simulink model "ami_fx_sbl_wide"  (R2012b)
(part 2 of 43)

      mask init:
      | gw_name = clear_name(gcb);
      | config.source = str2func('software_register_init');
      | config.toplevel = gcb;
      | xBlock( config, {io_dir, arith_type, bitwidth, bin_pt, ... 
      |     sample_period, gw_name, latency});
      mask TypeOptions io_dir: From Processor | To Processor
      mask TypeOptions arith_type: Unsigned | Signed  (2's comp)
  notused : xbsIndex_r4/Constant  const=0  gui_display_data_type=Fixed-point  arith_type=Boolean  n_bits=28  bin_pt=0  preci_type=Single  exp_width=8  frac_width=24  explicit_period=on  period=1  equ=P=C  opselect=C  inp2=PCIN>>17  opr=+  inp1=P  carry=CIN  dbl_ovrd=off  block_type=constant
  packetiser : Subsystem  mask{fft_bits=11}
      mask prompts: fft_bits "Number of frequencies (2^?)"
      mask help: Package 32 bit data into 64 bits and identify data as coming from antenna 0 or 1
  phase_invert1 : Subsystem
  phase_invert2 : Subsystem
  pipeline : Subsystem  AncestorBlock=casper_library_delays/pipeline  mask(pipeline){latency=1}
      mask help:
      | An explicitly laid-out delay line to avoid mapping to SRL16s
      | for use in pipelining to help achieve timing closure.
      mask init:
      | pipeline_init(gcb,'latency',latency);
      settings: AttributesFormatString=Latency = %<latency>
      mask Display:
      | port_label('input', 1, 'd');
      | port_label('output', 1, 'q');
      | disp(['Z^-', num2str(latency)]);
  pipeline1 : Subsystem  AncestorBlock=casper_library_delays/pipeline  mask(pipeline){latency=1}
      mask help:
      | An explicitly laid-out delay line to avoid mapping to SRL16s
      | for use in pipelining to help achieve timing closure.
      mask init:
      | pipeline_init(gcb,'latency',latency);
      settings: AttributesFormatString=Latency = %<latency>
      mask Display:
      | port_label('input', 1, 'd');
      | port_label('output', 1, 'q');
      | disp(['Z^-', num2str(latency)]);
  pipeline10 : Subsystem  AncestorBlock=casper_library_delays/pipeline  mask(pipeline){latency=3}
      mask help:
      | An explicitly laid-out delay line to avoid mapping to SRL16s
      | for use in pipelining to help achieve timing closure.
      mask init:
      | pipeline_init(gcb,'latency',latency);
      settings: AttributesFormatString=Latency = %<latency>
      mask Display:
      | port_label('input', 1, 'd');
      | port_label('output', 1, 'q');
      | disp(['Z^-', num2str(latency)]);
  pipeline100 : Subsystem  AncestorBlock=casper_library_delays/pipeline  mask(pipeline){latency=2}
      mask help:
      | An explicitly laid-out delay line to avoid mapping to SRL16s
      | for use in pipelining to help achieve timing closure.
      mask init:
      | pipeline_init(gcb,'latency',latency);
      settings: AttributesFormatString=Latency = %<latency>
      mask Display:
      | port_label('input', 1, 'd');
      | port_label('output', 1, 'q');
      | disp(['Z^-', num2str(latency)]);
  pipeline101 : Subsystem  AncestorBlock=casper_library_delays/pipeline  mask(pipeline){latency=2}
      mask help:
      | An explicitly laid-out delay line to avoid mapping to SRL16s
      | for use in pipelining to help achieve timing closure.
      mask init:
      | pipeline_init(gcb,'latency',latency);
      settings: AttributesFormatString=Latency = %<latency>
      mask Display:
      | port_label('input', 1, 'd');
      | port_label('output', 1, 'q');
      | disp(['Z^-', num2str(latency)]);
  pipeline102 : Subsystem  AncestorBlock=casper_library_delays/pipeline  mask(pipeline){latency=2}
      mask help:
      | An explicitly laid-out delay line to avoid mapping to SRL16s
      | for use in pipelining to help achieve timing closure.
      mask init:
      | pipeline_init(gcb,'latency',latency);
      settings: AttributesFormatString=Latency = %<latency>
      mask Display:
      | port_label('input', 1, 'd');
      | port_label('output', 1, 'q');
      | disp(['Z^-', num2str(latency)]);
  pipeline103 : Subsystem  AncestorBlock=casper_library_delays/pipeline  mask(pipeline){latency=2}
      mask help:
      | An explicitly laid-out delay line to avoid mapping to SRL16s
      | for use in pipelining to help achieve timing closure.
      mask init:
      | pipeline_init(gcb,'latency',latency);
      settings: AttributesFormatString=Latency = %<latency>
      mask Display:
      | port_label('input', 1, 'd');
      | port_label('output', 1, 'q');
      | disp(['Z^-', num2str(latency)]);
  pipeline104 : Subsystem  AncestorBlock=casper_library_delays/pipeline  mask(pipeline){latency=2}
      mask help:
      | An explicitly laid-out delay line to avoid mapping to SRL16s
      | for use in pipelining to help achieve timing closure.
      mask init:
      | pipeline_init(gcb,'latency',latency);
      settings: AttributesFormatString=Latency = %<latency>
      mask Display:
      | port_label('input', 1, 'd');
      | port_label('output', 1, 'q');
      | disp(['Z^-', num2str(latency)]);
  pipeline105 : Subsystem  AncestorBlock=casper_library_delays/pipeline  mask(pipeline){latency=2}
      mask help:
      | An explicitly laid-out delay line to avoid mapping to SRL16s
      | for use in pipelining to help achieve timing closure.
      mask init:
      | pipeline_init(gcb,'latency',latency);
      settings: AttributesFormatString=Latency = %<latency>
      mask Display:
      | port_label('input', 1, 'd');
      | port_label('output', 1, 'q');
      | disp(['Z^-', num2str(latency)]);
  pipeline106 : Subsystem  AncestorBlock=casper_library_delays/pipeline  mask(pipeline){latency=2}
      mask help:
      | An explicitly laid-out delay line to avoid mapping to SRL16s
      | for use in pipelining to help achieve timing closure.
      mask init:
      | pipeline_init(gcb,'latency',latency);
      settings: AttributesFormatString=Latency = %<latency>
      mask Display:
      | port_label('input', 1, 'd');
      | port_label('output', 1, 'q');
      | disp(['Z^-', num2str(latency)]);
  pipeline107 : Subsystem  AncestorBlock=casper_library_delays/pipeline  mask(pipeline){latency=2}
      mask help:
      | An explicitly laid-out delay line to avoid mapping to SRL16s
      | for use in pipelining to help achieve timing closure.
      mask init:
      | pipeline_init(gcb,'latency',latency);
      settings: AttributesFormatString=Latency = %<latency>
      mask Display:
      | port_label('input', 1, 'd');
      | port_label('output', 1, 'q');
      | disp(['Z^-', num2str(latency)]);
  pipeline108 : Subsystem  AncestorBlock=casper_library_delays/pipeline  mask(pipeline){latency=2}
      mask help:
      | An explicitly laid-out delay line to avoid mapping to SRL16s
      | for use in pipelining to help achieve timing closure.
      mask init:
      | pipeline_init(gcb,'latency',latency);
      settings: AttributesFormatString=Latency = %<latency>
      mask Display:
      | port_label('input', 1, 'd');
      | port_label('output', 1, 'q');
      | disp(['Z^-', num2str(latency)]);
  pipeline109 : Subsystem  AncestorBlock=casper_library_delays/pipeline  mask(pipeline){latency=2}
      mask help:
      | An explicitly laid-out delay line to avoid mapping to SRL16s
      | for use in pipelining to help achieve timing closure.
      mask init:
      | pipeline_init(gcb,'latency',latency);
      settings: AttributesFormatString=Latency = %<latency>
      mask Display:
      | port_label('input', 1, 'd');
      | port_label('output', 1, 'q');
      | disp(['Z^-', num2str(latency)]);
  pipeline11 : Subsystem  AncestorBlock=casper_library_delays/pipeline  mask(pipeline){latency=1}
      mask help:
      | An explicitly laid-out delay line to avoid mapping to SRL16s
      | for use in pipelining to help achieve timing closure.
      mask init:
      | pipeline_init(gcb,'latency',latency);
      settings: AttributesFormatString=Latency = %<latency>
      mask Display:
      | port_label('input', 1, 'd');
      | port_label('output', 1, 'q');
      | disp(['Z^-', num2str(latency)]);
  pipeline110 : Subsystem  AncestorBlock=casper_library_delays/pipeline  mask(pipeline){latency=2}
      mask help:
      | An explicitly laid-out delay line to avoid mapping to SRL16s
      | for use in pipelining to help achieve timing closure.
      mask init:
      | pipeline_init(gcb,'latency',latency);
      settings: AttributesFormatString=Latency = %<latency>
      mask Display:
      | port_label('input', 1, 'd');
      | port_label('output', 1, 'q');
      | disp(['Z^-', num2str(latency)]);
  pipeline12 : Subsystem  AncestorBlock=casper_library_delays/pipeline  mask(pipeline){latency=3}
      mask help:
      | An explicitly laid-out delay line to avoid mapping to SRL16s
      | for use in pipelining to help achieve timing closure.
      mask init:
      | pipeline_init(gcb,'latency',latency);
      settings: AttributesFormatString=Latency = %<latency>
      mask Display:
      | port_label('input', 1, 'd');
      | port_label('output', 1, 'q');
      | disp(['Z^-', num2str(latency)]);
  pipeline13 : Subsystem  AncestorBlock=casper_library_delays/pipeline  mask(pipeline){latency=1}
      mask help:
      | An explicitly laid-out delay line to avoid mapping to SRL16s
      | for use in pipelining to help achieve timing closure.
      mask init:
      | pipeline_init(gcb,'latency',latency);
      settings: AttributesFormatString=Latency = %<latency>
      mask Display:
      | port_label('input', 1, 'd');
      | port_label('output', 1, 'q');
      | disp(['Z^-', num2str(latency)]);
  pipeline14 : Subsystem  AncestorBlock=casper_library_delays/pipeline  mask(pipeline){latency=2}
      mask help:
      | An explicitly laid-out delay line to avoid mapping to SRL16s
      | for use in pipelining to help achieve timing closure.
      mask init:
      | pipeline_init(gcb,'latency',latency);
      settings: AttributesFormatString=Latency = %<latency>
      mask Display:
      | port_label('input', 1, 'd');
      | port_label('output', 1, 'q');
      | disp(['Z^-', num2str(latency)]);
  pipeline15 : Subsystem  AncestorBlock=casper_library_delays/pipeline  mask(pipeline){latency=2}
      mask help:
      | An explicitly laid-out delay line to avoid mapping to SRL16s
      | for use in pipelining to help achieve timing closure.
      mask init:
      | pipeline_init(gcb,'latency',latency);
      settings: AttributesFormatString=Latency = %<latency>
      mask Display:
      | port_label('input', 1, 'd');
      | port_label('output', 1, 'q');
      | disp(['Z^-', num2str(latency)]);
  pipeline16 : Subsystem  AncestorBlock=casper_library_delays/pipeline  mask(pipeline){latency=2}
      mask help:
      | An explicitly laid-out delay line to avoid mapping to SRL16s
      | for use in pipelining to help achieve timing closure.
      mask init:
      | pipeline_init(gcb,'latency',latency);
      settings: AttributesFormatString=Latency = %<latency>
      mask Display:
      | port_label('input', 1, 'd');
      | port_label('output', 1, 'q');
      | disp(['Z^-', num2str(latency)]);
  pipeline17 : Subsystem  AncestorBlock=casper_library_delays/pipeline  mask(pipeline){latency=2}
      mask help:
      | An explicitly laid-out delay line to avoid mapping to SRL16s
      | for use in pipelining to help achieve timing closure.
      mask init:
      | pipeline_init(gcb,'latency',latency);
      settings: AttributesFormatString=Latency = %<latency>
      mask Display:
      | port_label('input', 1, 'd');
      | port_label('output', 1, 'q');
      | disp(['Z^-', num2str(latency)]);
  pipeline18 : Subsystem  AncestorBlock=casper_library_delays/pipeline  mask(pipeline){latency=2}
      mask help:
      | An explicitly laid-out delay line to avoid mapping to SRL16s
      | for use in pipelining to help achieve timing closure.
      mask init:
      | pipeline_init(gcb,'latency',latency);
      settings: AttributesFormatString=Latency = %<latency>
      mask Display:
      | port_label('input', 1, 'd');
      | port_label('output', 1, 'q');
      | disp(['Z^-', num2str(latency)]);
  pipeline19 : Subsystem  AncestorBlock=casper_library_delays/pipeline  mask(pipeline){latency=1}
      mask help:
      | An explicitly laid-out delay line to avoid mapping to SRL16s
      | for use in pipelining to help achieve timing closure.
      mask init:
      | pipeline_init(gcb,'latency',latency);
      settings: AttributesFormatString=Latency = %<latency>
      mask Display:
      | port_label('input', 1, 'd');
      | port_label('output', 1, 'q');
      | disp(['Z^-', num2str(latency)]);
  pipeline2 : Subsystem  AncestorBlock=casper_library_delays/pipeline  mask(pipeline){latency=1}
      mask help:
      | An explicitly laid-out delay line to avoid mapping to SRL16s
      | for use in pipelining to help achieve timing closure.
      mask init:
      | pipeline_init(gcb,'latency',latency);
      settings: AttributesFormatString=Latency = %<latency>
      mask Display:
      | port_label('input', 1, 'd');
      | port_label('output', 1, 'q');
      | disp(['Z^-', num2str(latency)]);
  pipeline20 : Subsystem  AncestorBlock=casper_library_delays/pipeline  mask(pipeline){latency=1}
      mask help:
      | An explicitly laid-out delay line to avoid mapping to SRL16s
      | for use in pipelining to help achieve timing closure.
      mask init:
      | pipeline_init(gcb,'latency',latency);
      settings: AttributesFormatString=Latency = %<latency>
      mask Display:
      | port_label('input', 1, 'd');
      | port_label('output', 1, 'q');
      | disp(['Z^-', num2str(latency)]);
  pipeline21 : Subsystem  AncestorBlock=casper_library_delays/pipeline  mask(pipeline){latency=1}
      mask help:
      | An explicitly laid-out delay line to avoid mapping to SRL16s
      | for use in pipelining to help achieve timing closure.
      mask init:
      | pipeline_init(gcb,'latency',latency);
      settings: AttributesFormatString=Latency = %<latency>
      mask Display:
      | port_label('input', 1, 'd');
      | port_label('output', 1, 'q');
      | disp(['Z^-', num2str(latency)]);
  pipeline22 : Subsystem  AncestorBlock=casper_library_delays/pipeline  mask(pipeline){latency=1}
      mask help:
      | An explicitly laid-out delay line to avoid mapping to SRL16s
      | for use in pipelining to help achieve timing closure.
      mask init:
      | pipeline_init(gcb,'latency',latency);
      settings: AttributesFormatString=Latency = %<latency>
      mask Display:
      | port_label('input', 1, 'd');
      | port_label('output', 1, 'q');
      | disp(['Z^-', num2str(latency)]);
  pipeline23 : Subsystem  AncestorBlock=casper_library_delays/pipeline  mask(pipeline){latency=1}
      mask help:
      | An explicitly laid-out delay line to avoid mapping to SRL16s
      | for use in pipelining to help achieve timing closure.
      mask init:
      | pipeline_init(gcb,'latency',latency);
      settings: AttributesFormatString=Latency = %<latency>
      mask Display:
      | port_label('input', 1, 'd');
      | port_label('output', 1, 'q');
      | disp(['Z^-', num2str(latency)]);
  pipeline24 : Subsystem  AncestorBlock=casper_library_delays/pipeline  mask(pipeline){latency=1}
      mask help:
      | An explicitly laid-out delay line to avoid mapping to SRL16s
      | for use in pipelining to help achieve timing closure.
      mask init:
      | pipeline_init(gcb,'latency',latency);
      settings: AttributesFormatString=Latency = %<latency>
      mask Display:
      | port_label('input', 1, 'd');
      | port_label('output', 1, 'q');
      | disp(['Z^-', num2str(latency)]);
  pipeline25 : Subsystem  AncestorBlock=casper_library_delays/pipeline  mask(pipeline){latency=1}
      mask help:
      | An explicitly laid-out delay line to avoid mapping to SRL16s
      | for use in pipelining to help achieve timing closure.
      mask init:
      | pipeline_init(gcb,'latency',latency);
      settings: AttributesFormatString=Latency = %<latency>
      mask Display:
      | port_label('input', 1, 'd');
      | port_label('output', 1, 'q');
      | disp(['Z^-', num2str(latency)]);
  pipeline26 : Subsystem  AncestorBlock=casper_library_delays/pipeline  mask(pipeline){latency=1}
      mask help:
      | An explicitly laid-out delay line to avoid mapping to SRL16s
      | for use in pipelining to help achieve timing closure.
      mask init:
      | pipeline_init(gcb,'latency',latency);
      settings: AttributesFormatString=Latency = %<latency>
      mask Display:
      | port_label('input', 1, 'd');
      | port_label('output', 1, 'q');
      | disp(['Z^-', num2str(latency)]);
  pipeline27 : Subsystem  AncestorBlock=casper_library_delays/pipeline  mask(pipeline){latency=1}
      mask help:
      | An explicitly laid-out delay line to avoid mapping to SRL16s
      | for use in pipelining to help achieve timing closure.
      mask init:
      | pipeline_init(gcb,'latency',latency);
      settings: AttributesFormatString=Latency = %<latency>
      mask Display:
      | port_label('input', 1, 'd');
      | port_label('output', 1, 'q');
      | disp(['Z^-', num2str(latency)]);
  pipeline28 : Subsystem  AncestorBlock=casper_library_delays/pipeline  mask(pipeline){latency=1}
      mask help:
      | An explicitly laid-out delay line to avoid mapping to SRL16s
      | for use in pipelining to help achieve timing closure.
      mask init:
      | pipeline_init(gcb,'latency',latency);
      settings: AttributesFormatString=Latency = %<latency>
      mask Display:
      | port_label('input', 1, 'd');
      | port_label('output', 1, 'q');
      | disp(['Z^-', num2str(latency)]);
  pipeline29 : Subsystem  AncestorBlock=casper_library_delays/pipeline  mask(pipeline){latency=1}
      mask help:
      | An explicitly laid-out delay line to avoid mapping to SRL16s
      | for use in pipelining to help achieve timing closure.
      mask init:
      | pipeline_init(gcb,'latency',latency);
      settings: AttributesFormatString=Latency = %<latency>
      mask Display:
      | port_label('input', 1, 'd');
      | port_label('output', 1, 'q');
      | disp(['Z^-', num2str(latency)]);
  pipeline3 : Subsystem  AncestorBlock=casper_library_delays/pipeline  mask(pipeline){latency=1}
      mask help:
      | An explicitly laid-out delay line to avoid mapping to SRL16s
      | for use in pipelining to help achieve timing closure.
      mask init:
      | pipeline_init(gcb,'latency',latency);
      settings: AttributesFormatString=Latency = %<latency>
      mask Display:
      | port_label('input', 1, 'd');
      | port_label('output', 1, 'q');
      | disp(['Z^-', num2str(latency)]);
  pipeline30 : Subsystem  AncestorBlock=casper_library_delays/pipeline  mask(pipeline){latency=1}
      mask help:
      | An explicitly laid-out delay line to avoid mapping to SRL16s
      | for use in pipelining to help achieve timing closure.
      mask init:
      | pipeline_init(gcb,'latency',latency);
      settings: AttributesFormatString=Latency = %<latency>
      mask Display:
      | port_label('input', 1, 'd');
      | port_label('output', 1, 'q');
      | disp(['Z^-', num2str(latency)]);
  pipeline31 : Subsystem  AncestorBlock=casper_library_delays/pipeline  mask(pipeline){latency=1}
      mask help:
      | An explicitly laid-out delay line to avoid mapping to SRL16s
      | for use in pipelining to help achieve timing closure.
      mask init:
      | pipeline_init(gcb,'latency',latency);
      settings: AttributesFormatString=Latency = %<latency>
      mask Display:
      | port_label('input', 1, 'd');
      | port_label('output', 1, 'q');
      | disp(['Z^-', num2str(latency)]);
  pipeline32 : Subsystem  AncestorBlock=casper_library_delays/pipeline  mask(pipeline){latency=1}
      mask help:
      | An explicitly laid-out delay line to avoid mapping to SRL16s
      | for use in pipelining to help achieve timing closure.
      mask init:
      | pipeline_init(gcb,'latency',latency);
      settings: AttributesFormatString=Latency = %<latency>
      mask Display:
      | port_label('input', 1, 'd');
      | port_label('output', 1, 'q');
      | disp(['Z^-', num2str(latency)]);
  pipeline33 : Subsystem  AncestorBlock=casper_library_delays/pipeline  mask(pipeline){latency=1}
      mask help:
      | An explicitly laid-out delay line to avoid mapping to SRL16s
      | for use in pipelining to help achieve timing closure.
      mask init:
      | pipeline_init(gcb,'latency',latency);
      settings: AttributesFormatString=Latency = %<latency>
      mask Display:
      | port_label('input', 1, 'd');
      | port_label('output', 1, 'q');
      | disp(['Z^-', num2str(latency)]);
  pipeline34 : Subsystem  AncestorBlock=casper_library_delays/pipeline  mask(pipeline){latency=1}
      mask help:
      | An explicitly laid-out delay line to avoid mapping to SRL16s
      | for use in pipelining to help achieve timing closure.
      mask init:
      | pipeline_init(gcb,'latency',latency);
      settings: AttributesFormatString=Latency = %<latency>
      mask Display:
      | port_label('input', 1, 'd');
      | port_label('output', 1, 'q');
      | disp(['Z^-', num2str(latency)]);
  pipeline35 : Subsystem  AncestorBlock=casper_library_delays/pipeline  mask(pipeline){latency=1}
      mask help:
      | An explicitly laid-out delay line to avoid mapping to SRL16s
      | for use in pipelining to help achieve timing closure.
      mask init:
      | pipeline_init(gcb,'latency',latency);
      settings: AttributesFormatString=Latency = %<latency>
      mask Display:
      | port_label('input', 1, 'd');
      | port_label('output', 1, 'q');
      | disp(['Z^-', num2str(latency)]);
  pipeline36 : Subsystem  AncestorBlock=casper_library_delays/pipeline  mask(pipeline){latency=1}
      mask help:
      | An explicitly laid-out delay line to avoid mapping to SRL16s
      | for use in pipelining to help achieve timing closure.
      mask init:
      | pipeline_init(gcb,'latency',latency);
      settings: AttributesFormatString=Latency = %<latency>
      mask Display:
      | port_label('input', 1, 'd');
      | port_label('output', 1, 'q');
      | disp(['Z^-', num2str(latency)]);
  pipeline37 : Subsystem  AncestorBlock=casper_library_delays/pipeline  mask(pipeline){latency=1}
      mask help:
      | An explicitly laid-out delay line to avoid mapping to SRL16s
      | for use in pipelining to help achieve timing closure.
      mask init:
      | pipeline_init(gcb,'latency',latency);
      settings: AttributesFormatString=Latency = %<latency>
      mask Display:
      | port_label('input', 1, 'd');
      | port_label('output', 1, 'q');
      | disp(['Z^-', num2str(latency)]);
  pipeline38 : Subsystem  AncestorBlock=casper_library_delays/pipeline  mask(pipeline){latency=3}
      mask help:
      | An explicitly laid-out delay line to avoid mapping to SRL16s
      | for use in pipelining to help achieve timing closure.
      mask init:
      | pipeline_init(gcb,'latency',latency);
      settings: AttributesFormatString=Latency = %<latency>
      mask Display:
      | port_label('input', 1, 'd');
      | port_label('output', 1, 'q');
      | disp(['Z^-', num2str(latency)]);
  pipeline39 : Subsystem  AncestorBlock=casper_library_delays/pipeline  mask(pipeline){latency=1}
      mask help:
      | An explicitly laid-out delay line to avoid mapping to SRL16s
      | for use in pipelining to help achieve timing closure.
      mask init:
      | pipeline_init(gcb,'latency',latency);
      settings: AttributesFormatString=Latency = %<latency>
      mask Display:
      | port_label('input', 1, 'd');
      | port_label('output', 1, 'q');
      | disp(['Z^-', num2str(latency)]);
  pipeline4 : Subsystem  AncestorBlock=casper_library_delays/pipeline  mask(pipeline){latency=1}
      mask help:
      | An explicitly laid-out delay line to avoid mapping to SRL16s
      | for use in pipelining to help achieve timing closure.
      mask init:
      | pipeline_init(gcb,'latency',latency);
      settings: AttributesFormatString=Latency = %<latency>
      mask Display:
      | port_label('input', 1, 'd');
      | port_label('output', 1, 'q');
      | disp(['Z^-', num2str(latency)]);
  pipeline40 : Subsystem  AncestorBlock=casper_library_delays/pipeline  mask(pipeline){latency=1}
      mask help:
      | An explicitly laid-out delay line to avoid mapping to SRL16s
      | for use in pipelining to help achieve timing closure.
      mask init:
      | pipeline_init(gcb,'latency',latency);
      settings: AttributesFormatString=Latency = %<latency>
      mask Display:
      | port_label('input', 1, 'd');
      | port_label('output', 1, 'q');
      | disp(['Z^-', num2str(latency)]);
  pipeline41 : Subsystem  AncestorBlock=casper_library_delays/pipeline  mask(pipeline){latency=1}
      mask help:
      | An explicitly laid-out delay line to avoid mapping to SRL16s
      | for use in pipelining to help achieve timing closure.
      mask init:
      | pipeline_init(gcb,'latency',latency);
      settings: AttributesFormatString=Latency = %<latency>
      mask Display:
      | port_label('input', 1, 'd');
      | port_label('output', 1, 'q');
      | disp(['Z^-', num2str(latency)]);
  pipeline42 : Subsystem  AncestorBlock=casper_library_delays/pipeline  mask(pipeline){latency=1}
      mask help:
      | An explicitly laid-out delay line to avoid mapping to SRL16s
      | for use in pipelining to help achieve timing closure.
      mask init:
      | pipeline_init(gcb,'latency',latency);
      settings: AttributesFormatString=Latency = %<latency>
      mask Display:
      | port_label('input', 1, 'd');
      | port_label('output', 1, 'q');
      | disp(['Z^-', num2str(latency)]);
  pipeline43 : Subsystem  AncestorBlock=casper_library_delays/pipeline  mask(pipeline){latency=3}
      mask help:
      | An explicitly laid-out delay line to avoid mapping to SRL16s
      | for use in pipelining to help achieve timing closure.
      mask init:
      | pipeline_init(gcb,'latency',latency);
      settings: AttributesFormatString=Latency = %<latency>
      mask Display:
      | port_label('input', 1, 'd');
      | port_label('output', 1, 'q');
      | disp(['Z^-', num2str(latency)]);
  pipeline44 : Subsystem  AncestorBlock=casper_library_delays/pipeline  mask(pipeline){latency=1}
      mask help:
      | An explicitly laid-out delay line to avoid mapping to SRL16s
      | for use in pipelining to help achieve timing closure.
      mask init:
      | pipeline_init(gcb,'latency',latency);
      settings: AttributesFormatString=Latency = %<latency>
      mask Display:
      | port_label('input', 1, 'd');
      | port_label('output', 1, 'q');
      | disp(['Z^-', num2str(latency)]);
  pipeline45 : Subsystem  AncestorBlock=casper_library_delays/pipeline  mask(pipeline){latency=1}
      mask help:
      | An explicitly laid-out delay line to avoid mapping to SRL16s
      | for use in pipelining to help achieve timing closure.
      mask init:
      | pipeline_init(gcb,'latency',latency);
      settings: AttributesFormatString=Latency = %<latency>
      mask Display:
      | port_label('input', 1, 'd');
      | port_label('output', 1, 'q');
      | disp(['Z^-', num2str(latency)]);
  pipeline46 : Subsystem  AncestorBlock=casper_library_delays/pipeline  mask(pipeline){latency=1}
      mask help:
      | An explicitly laid-out delay line to avoid mapping to SRL16s
      | for use in pipelining to help achieve timing closure.
      mask init:
      | pipeline_init(gcb,'latency',latency);
      settings: AttributesFormatString=Latency = %<latency>
      mask Display:
      | port_label('input', 1, 'd');
      | port_label('output', 1, 'q');
      | disp(['Z^-', num2str(latency)]);
  pipeline47 : Subsystem  AncestorBlock=casper_library_delays/pipeline  mask(pipeline){latency=2}
      mask help:
      | An explicitly laid-out delay line to avoid mapping to SRL16s
      | for use in pipelining to help achieve timing closure.
      mask init:
      | pipeline_init(gcb,'latency',latency);
      settings: AttributesFormatString=Latency = %<latency>
      mask Display:
      | port_label('input', 1, 'd');
      | port_label('output', 1, 'q');
      | disp(['Z^-', num2str(latency)]);
  pipeline48 : Subsystem  AncestorBlock=casper_library_delays/pipeline  mask(pipeline){latency=1}
      mask help:
      | An explicitly laid-out delay line to avoid mapping to SRL16s
      | for use in pipelining to help achieve timing closure.
      mask init:
      | pipeline_init(gcb,'latency',latency);
      settings: AttributesFormatString=Latency = %<latency>
      mask Display:
      | port_label('input', 1, 'd');
      | port_label('output', 1, 'q');
      | disp(['Z^-', num2str(latency)]);
  pipeline49 : Subsystem  AncestorBlock=casper_library_delays/pipeline  mask(pipeline){latency=1}
      mask help:
      | An explicitly laid-out delay line to avoid mapping to SRL16s
      | for use in pipelining to help achieve timing closure.
      mask init:
      | pipeline_init(gcb,'latency',latency);
      settings: AttributesFormatString=Latency = %<latency>
      mask Display:
      | port_label('input', 1, 'd');
      | port_label('output', 1, 'q');
      | disp(['Z^-', num2str(latency)]);
  pipeline5 : Subsystem  AncestorBlock=casper_library_delays/pipeline  mask(pipeline){latency=1}
      mask help:
      | An explicitly laid-out delay line to avoid mapping to SRL16s
      | for use in pipelining to help achieve timing closure.
      mask init:
      | pipeline_init(gcb,'latency',latency);
      settings: AttributesFormatString=Latency = %<latency>
      mask Display:
      | port_label('input', 1, 'd');
      | port_label('output', 1, 'q');
      | disp(['Z^-', num2str(latency)]);
  pipeline50 : Subsystem  AncestorBlock=casper_library_delays/pipeline  mask(pipeline){latency=1}
      mask help:
      | An explicitly laid-out delay line to avoid mapping to SRL16s
      | for use in pipelining to help achieve timing closure.
      mask init:
      | pipeline_init(gcb,'latency',latency);
      settings: AttributesFormatString=Latency = %<latency>
      mask Display:
      | port_label('input', 1, 'd');
      | port_label('output', 1, 'q');
      | disp(['Z^-', num2str(latency)]);
  pipeline51 : Subsystem  AncestorBlock=casper_library_delays/pipeline  mask(pipeline){latency=1}
      mask help:
      | An explicitly laid-out delay line to avoid mapping to SRL16s
      | for use in pipelining to help achieve timing closure.
      mask init:
      | pipeline_init(gcb,'latency',latency);
      settings: AttributesFormatString=Latency = %<latency>
      mask Display:
      | port_label('input', 1, 'd');
      | port_label('output', 1, 'q');
      | disp(['Z^-', num2str(latency)]);
  pipeline52 : Subsystem  AncestorBlock=casper_library_delays/pipeline  mask(pipeline){latency=1}
      mask help:
      | An explicitly laid-out delay line to avoid mapping to SRL16s
      | for use in pipelining to help achieve timing closure.
      mask init:
      | pipeline_init(gcb,'latency',latency);
      settings: AttributesFormatString=Latency = %<latency>
      mask Display:
      | port_label('input', 1, 'd');
      | port_label('output', 1, 'q');
      | disp(['Z^-', num2str(latency)]);
  pipeline53 : Subsystem  AncestorBlock=casper_library_delays/pipeline  mask(pipeline){latency=1}
      mask help:
      | An explicitly laid-out delay line to avoid mapping to SRL16s
      | for use in pipelining to help achieve timing closure.
      mask init:
      | pipeline_init(gcb,'latency',latency);
      settings: AttributesFormatString=Latency = %<latency>
      mask Display:
      | port_label('input', 1, 'd');
      | port_label('output', 1, 'q');
      | disp(['Z^-', num2str(latency)]);
  pipeline54 : Subsystem  AncestorBlock=casper_library_delays/pipeline  mask(pipeline){latency=1}
      mask help:
      | An explicitly laid-out delay line to avoid mapping to SRL16s
      | for use in pipelining to help achieve timing closure.
      mask init:
      | pipeline_init(gcb,'latency',latency);
      settings: AttributesFormatString=Latency = %<latency>
      mask Display:
      | port_label('input', 1, 'd');
      | port_label('output', 1, 'q');
      | disp(['Z^-', num2str(latency)]);
  pipeline55 : Subsystem  AncestorBlock=casper_library_delays/pipeline  mask(pipeline){latency=1}
      mask help:
      | An explicitly laid-out delay line to avoid mapping to SRL16s
      | for use in pipelining to help achieve timing closure.
      mask init:
      | pipeline_init(gcb,'latency',latency);
      settings: AttributesFormatString=Latency = %<latency>
      mask Display:
      | port_label('input', 1, 'd');
      | port_label('output', 1, 'q');
      | disp(['Z^-', num2str(latency)]);
  pipeline56 : Subsystem  AncestorBlock=casper_library_delays/pipeline  mask(pipeline){latency=1}
      mask help:
      | An explicitly laid-out delay line to avoid mapping to SRL16s
      | for use in pipelining to help achieve timing closure.
      mask init:
      | pipeline_init(gcb,'latency',latency);
      settings: AttributesFormatString=Latency = %<latency>
      mask Display:
      | port_label('input', 1, 'd');
      | port_label('output', 1, 'q');
      | disp(['Z^-', num2str(latency)]);
  pipeline57 : Subsystem  AncestorBlock=casper_library_delays/pipeline  mask(pipeline){latency=1}
      mask help:
      | An explicitly laid-out delay line to avoid mapping to SRL16s
      | for use in pipelining to help achieve timing closure.
      mask init:
      | pipeline_init(gcb,'latency',latency);
      settings: AttributesFormatString=Latency = %<latency>
      mask Display:
      | port_label('input', 1, 'd');
      | port_label('output', 1, 'q');
      | disp(['Z^-', num2str(latency)]);
  pipeline58 : Subsystem  AncestorBlock=casper_library_delays/pipeline  mask(pipeline){latency=2}
      mask help:
      | An explicitly laid-out delay line to avoid mapping to SRL16s
      | for use in pipelining to help achieve timing closure.
      mask init:
      | pipeline_init(gcb,'latency',latency);
      settings: AttributesFormatString=Latency = %<latency>
      mask Display:
      | port_label('input', 1, 'd');
      | port_label('output', 1, 'q');
      | disp(['Z^-', num2str(latency)]);
  pipeline59 : Subsystem  AncestorBlock=casper_library_delays/pipeline  mask(pipeline){latency=1}
      mask help:
      | An explicitly laid-out delay line to avoid mapping to SRL16s
      | for use in pipelining to help achieve timing closure.
      mask init:
      | pipeline_init(gcb,'latency',latency);
      settings: AttributesFormatString=Latency = %<latency>
      mask Display:
      | port_label('input', 1, 'd');
      | port_label('output', 1, 'q');
      | disp(['Z^-', num2str(latency)]);
  pipeline6 : Subsystem  AncestorBlock=casper_library_delays/pipeline  mask(pipeline){latency=1}
      mask help:
      | An explicitly laid-out delay line to avoid mapping to SRL16s
      | for use in pipelining to help achieve timing closure.
      mask init:
      | pipeline_init(gcb,'latency',latency);
      settings: AttributesFormatString=Latency = %<latency>
      mask Display:
      | port_label('input', 1, 'd');
      | port_label('output', 1, 'q');
      | disp(['Z^-', num2str(latency)]);
  pipeline60 : Subsystem  AncestorBlock=casper_library_delays/pipeline  mask(pipeline){latency=1}
      mask help:
      | An explicitly laid-out delay line to avoid mapping to SRL16s
      | for use in pipelining to help achieve timing closure.
      mask init:
      | pipeline_init(gcb,'latency',latency);
      settings: AttributesFormatString=Latency = %<latency>
      mask Display:
      | port_label('input', 1, 'd');
      | port_label('output', 1, 'q');
      | disp(['Z^-', num2str(latency)]);
  pipeline61 : Subsystem  AncestorBlock=casper_library_delays/pipeline  mask(pipeline){latency=1}
      mask help:
      | An explicitly laid-out delay line to avoid mapping to SRL16s
      | for use in pipelining to help achieve timing closure.
      mask init:
      | pipeline_init(gcb,'latency',latency);
      settings: AttributesFormatString=Latency = %<latency>
      mask Display:
      | port_label('input', 1, 'd');
      | port_label('output', 1, 'q');
      | disp(['Z^-', num2str(latency)]);
  pipeline62 : Subsystem  AncestorBlock=casper_library_delays/pipeline  mask(pipeline){latency=1}
      mask help:
      | An explicitly laid-out delay line to avoid mapping to SRL16s
      | for use in pipelining to help achieve timing closure.
      mask init:
      | pipeline_init(gcb,'latency',latency);
      settings: AttributesFormatString=Latency = %<latency>
      mask Display:
      | port_label('input', 1, 'd');
      | port_label('output', 1, 'q');
      | disp(['Z^-', num2str(latency)]);
  pipeline63 : Subsystem  AncestorBlock=casper_library_delays/pipeline  mask(pipeline){latency=1}
      mask help:
      | An explicitly laid-out delay line to avoid mapping to SRL16s
      | for use in pipelining to help achieve timing closure.
      mask init:
      | pipeline_init(gcb,'latency',latency);
      settings: AttributesFormatString=Latency = %<latency>
      mask Display:
      | port_label('input', 1, 'd');
      | port_label('output', 1, 'q');
      | disp(['Z^-', num2str(latency)]);
  pipeline64 : Subsystem  AncestorBlock=casper_library_delays/pipeline  mask(pipeline){latency=1}
      mask help:
      | An explicitly laid-out delay line to avoid mapping to SRL16s
      | for use in pipelining to help achieve timing closure.
      mask init:
      | pipeline_init(gcb,'latency',latency);
      settings: AttributesFormatString=Latency = %<latency>
      mask Display:
      | port_label('input', 1, 'd');
      | port_label('output', 1, 'q');
      | disp(['Z^-', num2str(latency)]);
  pipeline65 : Subsystem  AncestorBlock=casper_library_delays/pipeline  mask(pipeline){latency=1}
      mask help:
      | An explicitly laid-out delay line to avoid mapping to SRL16s
      | for use in pipelining to help achieve timing closure.
      mask init:
      | pipeline_init(gcb,'latency',latency);
      settings: AttributesFormatString=Latency = %<latency>
      mask Display:
      | port_label('input', 1, 'd');
      | port_label('output', 1, 'q');
      | disp(['Z^-', num2str(latency)]);
  pipeline66 : Subsystem  AncestorBlock=casper_library_delays/pipeline  mask(pipeline){latency=1}
      mask help:
      | An explicitly laid-out delay line to avoid mapping to SRL16s
      | for use in pipelining to help achieve timing closure.
      mask init:
      | pipeline_init(gcb,'latency',latency);
      settings: AttributesFormatString=Latency = %<latency>
      mask Display:
      | port_label('input', 1, 'd');
      | port_label('output', 1, 'q');
      | disp(['Z^-', num2str(latency)]);
  pipeline67 : Subsystem  AncestorBlock=casper_library_delays/pipeline  mask(pipeline){latency=1}
      mask help:
      | An explicitly laid-out delay line to avoid mapping to SRL16s
      | for use in pipelining to help achieve timing closure.
      mask init:
      | pipeline_init(gcb,'latency',latency);
      settings: AttributesFormatString=Latency = %<latency>
      mask Display:
      | port_label('input', 1, 'd');
      | port_label('output', 1, 'q');
      | disp(['Z^-', num2str(latency)]);
  pipeline68 : Subsystem  AncestorBlock=casper_library_delays/pipeline  mask(pipeline){latency=2}
      mask help:
      | An explicitly laid-out delay line to avoid mapping to SRL16s
      | for use in pipelining to help achieve timing closure.
      mask init:
      | pipeline_init(gcb,'latency',latency);
      settings: AttributesFormatString=Latency = %<latency>
      mask Display:
      | port_label('input', 1, 'd');
      | port_label('output', 1, 'q');
      | disp(['Z^-', num2str(latency)]);
  pipeline69 : Subsystem  AncestorBlock=casper_library_delays/pipeline  mask(pipeline){latency=1}
      mask help:
      | An explicitly laid-out delay line to avoid mapping to SRL16s
      | for use in pipelining to help achieve timing closure.
      mask init:
      | pipeline_init(gcb,'latency',latency);
      settings: AttributesFormatString=Latency = %<latency>
      mask Display:
      | port_label('input', 1, 'd');
      | port_label('output', 1, 'q');
      | disp(['Z^-', num2str(latency)]);
  pipeline7 : Subsystem  AncestorBlock=casper_library_delays/pipeline  mask(pipeline){latency=1}
      mask help:
      | An explicitly laid-out delay line to avoid mapping to SRL16s
      | for use in pipelining to help achieve timing closure.
      mask init:
      | pipeline_init(gcb,'latency',latency);
      settings: AttributesFormatString=Latency = %<latency>
      mask Display:
      | port_label('input', 1, 'd');
      | port_label('output', 1, 'q');
      | disp(['Z^-', num2str(latency)]);
  pipeline70 : Subsystem  AncestorBlock=casper_library_delays/pipeline  mask(pipeline){latency=1}
      mask help:
      | An explicitly laid-out delay line to avoid mapping to SRL16s
      | for use in pipelining to help achieve timing closure.
      mask init:
      | pipeline_init(gcb,'latency',latency);
      settings: AttributesFormatString=Latency = %<latency>
      mask Display:
      | port_label('input', 1, 'd');
      | port_label('output', 1, 'q');
      | disp(['Z^-', num2str(latency)]);
  pipeline71 : Subsystem  AncestorBlock=casper_library_delays/pipeline  mask(pipeline){latency=1}
      mask help:
      | An explicitly laid-out delay line to avoid mapping to SRL16s
      | for use in pipelining to help achieve timing closure.
      mask init:
      | pipeline_init(gcb,'latency',latency);
      settings: AttributesFormatString=Latency = %<latency>
      mask Display:
      | port_label('input', 1, 'd');
      | port_label('output', 1, 'q');
      | disp(['Z^-', num2str(latency)]);
  pipeline72 : Subsystem  AncestorBlock=casper_library_delays/pipeline  mask(pipeline){latency=1}
      mask help:
      | An explicitly laid-out delay line to avoid mapping to SRL16s
      | for use in pipelining to help achieve timing closure.
      mask init:
      | pipeline_init(gcb,'latency',latency);
      settings: AttributesFormatString=Latency = %<latency>
      mask Display:
      | port_label('input', 1, 'd');
      | port_label('output', 1, 'q');
      | disp(['Z^-', num2str(latency)]);
  pipeline73 : Subsystem  AncestorBlock=casper_library_delays/pipeline  mask(pipeline){latency=2}
      mask help:
      | An explicitly laid-out delay line to avoid mapping to SRL16s
      | for use in pipelining to help achieve timing closure.
      mask init:
      | pipeline_init(gcb,'latency',latency);
      settings: AttributesFormatString=Latency = %<latency>
      mask Display:
      | port_label('input', 1, 'd');
      | port_label('output', 1, 'q');
      | disp(['Z^-', num2str(latency)]);
  pipeline74 : Subsystem  AncestorBlock=casper_library_delays/pipeline  mask(pipeline){latency=2}
      mask help:
      | An explicitly laid-out delay line to avoid mapping to SRL16s
      | for use in pipelining to help achieve timing closure.
      mask init:
      | pipeline_init(gcb,'latency',latency);
      settings: AttributesFormatString=Latency = %<latency>
      mask Display:
      | port_label('input', 1, 'd');
      | port_label('output', 1, 'q');
      | disp(['Z^-', num2str(latency)]);
  pipeline75 : Subsystem  AncestorBlock=casper_library_delays/pipeline  mask(pipeline){latency=2}
      mask help:
      | An explicitly laid-out delay line to avoid mapping to SRL16s
      | for use in pipelining to help achieve timing closure.
      mask init:
      | pipeline_init(gcb,'latency',latency);
      settings: AttributesFormatString=Latency = %<latency>
      mask Display:
      | port_label('input', 1, 'd');
      | port_label('output', 1, 'q');
      | disp(['Z^-', num2str(latency)]);
  pipeline76 : Subsystem  AncestorBlock=casper_library_delays/pipeline  mask(pipeline){latency=1}
      mask help:
      | An explicitly laid-out delay line to avoid mapping to SRL16s
      | for use in pipelining to help achieve timing closure.
      mask init:
      | pipeline_init(gcb,'latency',latency);
      settings: AttributesFormatString=Latency = %<latency>
      mask Display:
      | port_label('input', 1, 'd');
      | port_label('output', 1, 'q');
      | disp(['Z^-', num2str(latency)]);
  pipeline77 : Subsystem  AncestorBlock=casper_library_delays/pipeline  mask(pipeline){latency=1}
      mask help:
      | An explicitly laid-out delay line to avoid mapping to SRL16s
      | for use in pipelining to help achieve timing closure.
      mask init:
      | pipeline_init(gcb,'latency',latency);
      settings: AttributesFormatString=Latency = %<latency>
      mask Display:
      | port_label('input', 1, 'd');
      | port_label('output', 1, 'q');
      | disp(['Z^-', num2str(latency)]);
  pipeline78 : Subsystem  AncestorBlock=casper_library_delays/pipeline  mask(pipeline){latency=1}
      mask help:
      | An explicitly laid-out delay line to avoid mapping to SRL16s
      | for use in pipelining to help achieve timing closure.
      mask init:
      | pipeline_init(gcb,'latency',latency);
      settings: AttributesFormatString=Latency = %<latency>
      mask Display:
      | port_label('input', 1, 'd');
      | port_label('output', 1, 'q');
      | disp(['Z^-', num2str(latency)]);
  pipeline79 : Subsystem  AncestorBlock=casper_library_delays/pipeline  mask(pipeline){latency=1}
      mask help:
      | An explicitly laid-out delay line to avoid mapping to SRL16s
      | for use in pipelining to help achieve timing closure.
      mask init:
      | pipeline_init(gcb,'latency',latency);
      settings: AttributesFormatString=Latency = %<latency>
      mask Display:
      | port_label('input', 1, 'd');
      | port_label('output', 1, 'q');
      | disp(['Z^-', num2str(latency)]);
  pipeline8 : Subsystem  AncestorBlock=casper_library_delays/pipeline  mask(pipeline){latency=1}
      mask help:
      | An explicitly laid-out delay line to avoid mapping to SRL16s
      | for use in pipelining to help achieve timing closure.
      mask init:
      | pipeline_init(gcb,'latency',latency);
      settings: AttributesFormatString=Latency = %<latency>
      mask Display:
      | port_label('input', 1, 'd');
      | port_label('output', 1, 'q');
      | disp(['Z^-', num2str(latency)]);
  pipeline80 : Subsystem  AncestorBlock=casper_library_delays/pipeline  mask(pipeline){latency=1}
      mask help:
      | An explicitly laid-out delay line to avoid mapping to SRL16s
      | for use in pipelining to help achieve timing closure.
      mask init:
      | pipeline_init(gcb,'latency',latency);
      settings: AttributesFormatString=Latency = %<latency>
      mask Display:
      | port_label('input', 1, 'd');
      | port_label('output', 1, 'q');
      | disp(['Z^-', num2str(latency)]);
  pipeline81 : Subsystem  AncestorBlock=casper_library_delays/pipeline  mask(pipeline){latency=1}
      mask help:
      | An explicitly laid-out delay line to avoid mapping to SRL16s
      | for use in pipelining to help achieve timing closure.
      mask init:
      | pipeline_init(gcb,'latency',latency);
      settings: AttributesFormatString=Latency = %<latency>
      mask Display:
      | port_label('input', 1, 'd');
      | port_label('output', 1, 'q');
      | disp(['Z^-', num2str(latency)]);
  pipeline82 : Subsystem  AncestorBlock=casper_library_delays/pipeline  mask(pipeline){latency=4}
      mask help:
      | An explicitly laid-out delay line to avoid mapping to SRL16s
      | for use in pipelining to help achieve timing closure.
      mask init:
      | pipeline_init(gcb,'latency',latency);
      settings: AttributesFormatString=Latency = %<latency>
      mask Display:
      | port_label('input', 1, 'd');
      | port_label('output', 1, 'q');
      | disp(['Z^-', num2str(latency)]);
  pipeline83 : Subsystem  AncestorBlock=casper_library_delays/pipeline  mask(pipeline){latency=4}
      mask help:
      | An explicitly laid-out delay line to avoid mapping to SRL16s
      | for use in pipelining to help achieve timing closure.
      mask init:
      | pipeline_init(gcb,'latency',latency);
      settings: AttributesFormatString=Latency = %<latency>
      mask Display:
      | port_label('input', 1, 'd');
      | port_label('output', 1, 'q');
      | disp(['Z^-', num2str(latency)]);
  pipeline84 : Subsystem  AncestorBlock=casper_library_delays/pipeline  mask(pipeline){latency=4}
      mask help:
      | An explicitly laid-out delay line to avoid mapping to SRL16s
      | for use in pipelining to help achieve timing closure.
      mask init:
      | pipeline_init(gcb,'latency',latency);
      settings: AttributesFormatString=Latency = %<latency>
      mask Display:
      | port_label('input', 1, 'd');
      | port_label('output', 1, 'q');
      | disp(['Z^-', num2str(latency)]);
  pipeline85 : Subsystem  AncestorBlock=casper_library_delays/pipeline  mask(pipeline){latency=4}
      mask help:
      | An explicitly laid-out delay line to avoid mapping to SRL16s
      | for use in pipelining to help achieve timing closure.
      mask init:
      | pipeline_init(gcb,'latency',latency);
      settings: AttributesFormatString=Latency = %<latency>
      mask Display:
      | port_label('input', 1, 'd');
      | port_label('output', 1, 'q');
      | disp(['Z^-', num2str(latency)]);
  pipeline86 : Subsystem  AncestorBlock=casper_library_delays/pipeline  mask(pipeline){latency=1}
      mask help:
      | An explicitly laid-out delay line to avoid mapping to SRL16s
      | for use in pipelining to help achieve timing closure.
      mask init:
      | pipeline_init(gcb,'latency',latency);
      settings: AttributesFormatString=Latency = %<latency>
      mask Display:
      | port_label('input', 1, 'd');
      | port_label('output', 1, 'q');
      | disp(['Z^-', num2str(latency)]);
  pipeline87 : Subsystem  AncestorBlock=casper_library_delays/pipeline  mask(pipeline){latency=4}
      mask help:
      | An explicitly laid-out delay line to avoid mapping to SRL16s
      | for use in pipelining to help achieve timing closure.
      mask init:
      | pipeline_init(gcb,'latency',latency);
      settings: AttributesFormatString=Latency = %<latency>
      mask Display:
      | port_label('input', 1, 'd');
      | port_label('output', 1, 'q');
      | disp(['Z^-', num2str(latency)]);
  pipeline88 : Subsystem  AncestorBlock=casper_library_delays/pipeline  mask(pipeline){latency=4}
      mask help:
      | An explicitly laid-out delay line to avoid mapping to SRL16s
      | for use in pipelining to help achieve timing closure.
      mask init:
      | pipeline_init(gcb,'latency',latency);
      settings: AttributesFormatString=Latency = %<latency>
      mask Display:
      | port_label('input', 1, 'd');
      | port_label('output', 1, 'q');
      | disp(['Z^-', num2str(latency)]);
  pipeline89 : Subsystem  AncestorBlock=casper_library_delays/pipeline  mask(pipeline){latency=1}
      mask help:
      | An explicitly laid-out delay line to avoid mapping to SRL16s
      | for use in pipelining to help achieve timing closure.
      mask init:
      | pipeline_init(gcb,'latency',latency);
      settings: AttributesFormatString=Latency = %<latency>
      mask Display:
      | port_label('input', 1, 'd');
      | port_label('output', 1, 'q');
      | disp(['Z^-', num2str(latency)]);
  pipeline9 : Subsystem  AncestorBlock=casper_library_delays/pipeline  mask(pipeline){latency=1}
      mask help:
      | An explicitly laid-out delay line to avoid mapping to SRL16s
      | for use in pipelining to help achieve timing closure.
      mask init:
      | pipeline_init(gcb,'latency',latency);
      settings: AttributesFormatString=Latency = %<latency>
      mask Display:
      | port_label('input', 1, 'd');
      | port_label('output', 1, 'q');
      | disp(['Z^-', num2str(latency)]);
  pipeline90 : Subsystem  AncestorBlock=casper_library_delays/pipeline  mask(pipeline){latency=1}
      mask help:
      | An explicitly laid-out delay line to avoid mapping to SRL16s
      | for use in pipelining to help achieve timing closure.
      mask init:
      | pipeline_init(gcb,'latency',latency);
      settings: AttributesFormatString=Latency = %<latency>
      mask Display:
      | port_label('input', 1, 'd');
      | port_label('output', 1, 'q');
      | disp(['Z^-', num2str(latency)]);
  pipeline91 : Subsystem  AncestorBlock=casper_library_delays/pipeline  mask(pipeline){latency=4}
      mask help:
      | An explicitly laid-out delay line to avoid mapping to SRL16s
      | for use in pipelining to help achieve timing closure.
      mask init:
      | pipeline_init(gcb,'latency',latency);
      settings: AttributesFormatString=Latency = %<latency>
      mask Display:
      | port_label('input', 1, 'd');
      | port_label('output', 1, 'q');
      | disp(['Z^-', num2str(latency)]);
  pipeline92 : Subsystem  AncestorBlock=casper_library_delays/pipeline  mask(pipeline){latency=2}
      mask help:
      | An explicitly laid-out delay line to avoid mapping to SRL16s
      | for use in pipelining to help achieve timing closure.
      mask init:
      | pipeline_init(gcb,'latency',latency);
      settings: AttributesFormatString=Latency = %<latency>
      mask Display:
      | port_label('input', 1, 'd');
      | port_label('output', 1, 'q');
      | disp(['Z^-', num2str(latency)]);
  pipeline93 : Subsystem  AncestorBlock=casper_library_delays/pipeline  mask(pipeline){latency=2}
      mask help:
      | An explicitly laid-out delay line to avoid mapping to SRL16s
      | for use in pipelining to help achieve timing closure.
      mask init:
      | pipeline_init(gcb,'latency',latency);
      settings: AttributesFormatString=Latency = %<latency>
      mask Display:
      | port_label('input', 1, 'd');
      | port_label('output', 1, 'q');
      | disp(['Z^-', num2str(latency)]);
  pipeline94 : Subsystem  AncestorBlock=casper_library_delays/pipeline  mask(pipeline){latency=2}
      mask help:
      | An explicitly laid-out delay line to avoid mapping to SRL16s
      | for use in pipelining to help achieve timing closure.
      mask init:
      | pipeline_init(gcb,'latency',latency);
      settings: AttributesFormatString=Latency = %<latency>
      mask Display:
      | port_label('input', 1, 'd');
      | port_label('output', 1, 'q');
      | disp(['Z^-', num2str(latency)]);
  pipeline95 : Subsystem  AncestorBlock=casper_library_delays/pipeline  mask(pipeline){latency=2}
      mask help:
      | An explicitly laid-out delay line to avoid mapping to SRL16s
      | for use in pipelining to help achieve timing closure.
      mask init:
      | pipeline_init(gcb,'latency',latency);
      settings: AttributesFormatString=Latency = %<latency>
      mask Display:
      | port_label('input', 1, 'd');
      | port_label('output', 1, 'q');
      | disp(['Z^-', num2str(latency)]);
  pipeline96 : Subsystem  AncestorBlock=casper_library_delays/pipeline  mask(pipeline){latency=2}
      mask help:
      | An explicitly laid-out delay line to avoid mapping to SRL16s
      | for use in pipelining to help achieve timing closure.
      mask init:
      | pipeline_init(gcb,'latency',latency);
      settings: AttributesFormatString=Latency = %<latency>
      mask Display:
      | port_label('input', 1, 'd');
      | port_label('output', 1, 'q');
      | disp(['Z^-', num2str(latency)]);
  pipeline97 : Subsystem  AncestorBlock=casper_library_delays/pipeline  mask(pipeline){latency=2}
      mask help:
      | An explicitly laid-out delay line to avoid mapping to SRL16s
      | for use in pipelining to help achieve timing closure.
      mask init:
      | pipeline_init(gcb,'latency',latency);
      settings: AttributesFormatString=Latency = %<latency>
      mask Display:
      | port_label('input', 1, 'd');
      | port_label('output', 1, 'q');
      | disp(['Z^-', num2str(latency)]);
  pipeline98 : Subsystem  AncestorBlock=casper_library_delays/pipeline  mask(pipeline){latency=2}
      mask help:
      | An explicitly laid-out delay line to avoid mapping to SRL16s
      | for use in pipelining to help achieve timing closure.
      mask init:
      | pipeline_init(gcb,'latency',latency);
      settings: AttributesFormatString=Latency = %<latency>
      mask Display:
      | port_label('input', 1, 'd');
      | port_label('output', 1, 'q');
      | disp(['Z^-', num2str(latency)]);
  pipeline99 : Subsystem  AncestorBlock=casper_library_delays/pipeline  mask(pipeline){latency=2}
      mask help:
      | An explicitly laid-out delay line to avoid mapping to SRL16s
      | for use in pipelining to help achieve timing closure.
      mask init:
      | pipeline_init(gcb,'latency',latency);
      settings: AttributesFormatString=Latency = %<latency>
      mask Display:
      | port_label('input', 1, 'd');
      | port_label('output', 1, 'q');
      | disp(['Z^-', num2str(latency)]);
  posedge1 : Subsystem  AncestorBlock=casper_library_misc/edge_detect  mask(edge_detect){edge=Rising, polarity=Active High, x_in=[0 0.08 0.08 0.16 0.16 0.24 0.24 0.32 0.32 0.4], y_in=[-1 -1  1  1  1  1  1  1  1  1], x_out=[0.6 0.68 0.68 0.76 0.76 0.84 0.84 0.92 0.92 1], y_out=[-1 -1  1  1 -1 -1 -1 -1 -1 -1]}
      mask prompts: edge "Edge Type"; polarity "Output Polarity"; x_in "Input X Positions"; y_in "Input Y Positions"; x_out "Output X Positions"; y_out "Output Y Positions"
      mask help: Output is active for one-cycle after each edge of the specified type (i.e. rising, falling or both).
      mask init: same as ami_fx_sbl_wide/edge_detect
      settings: AttributesFormatString=|
      | rising edges
      | active high
      mask Help: Output is active for one-cycle after each edge of the specified type (i.e. rising, falling, or both).  Latency is zero.
      mask TypeOptions edge: Rising | Falling | Both
      mask TypeOptions polarity: Active High | Active Low
      mask Display:
      | plot(x_in_num,0.5+y_in_num*0.2);
      | plot(x_out_num,0.5+y_out_num*0.2);
  posedge2 : Subsystem  AncestorBlock=casper_library_misc/edge_detect  mask(edge_detect){edge=Rising, polarity=Active High, x_in=[0 0.08 0.08 0.16 0.16 0.24 0.24 0.32 0.32 0.4], y_in=[-1 -1  1  1  1  1  1  1  1  1], x_out=[0.6 0.68 0.68 0.76 0.76 0.84 0.84 0.92 0.92 1], y_out=[-1 -1  1  1 -1 -1 -1 -1 -1 -1]}
      mask prompts: edge "Edge Type"; polarity "Output Polarity"; x_in "Input X Positions"; y_in "Input Y Positions"; x_out "Output X Positions"; y_out "Output Y Positions"
      mask help: Output is active for one-cycle after each edge of the specified type (i.e. rising, falling or both).
      mask init: same as ami_fx_sbl_wide/edge_detect
      settings: AttributesFormatString=|
      | rising edges
      | active high
      mask Help: Output is active for one-cycle after each edge of the specified type (i.e. rising, falling, or both).  Latency is zero.
      mask TypeOptions edge: Rising | Falling | Both
      mask TypeOptions polarity: Active High | Active Low
      mask Display:
      | plot(x_in_num,0.5+y_in_num*0.2);
      | plot(x_out_num,0.5+y_out_num*0.2);
  posedge23 : Subsystem  AncestorBlock=casper_library_misc/edge_detect  mask(edge_detect){edge=Rising, polarity=Active High, x_in=[0 0.08 0.08 0.16 0.16 0.24 0.24 0.32 0.32 0.4], y_in=[-1 -1  1  1  1  1  1  1  1  1], x_out=[0.6 0.68 0.68 0.76 0.76 0.84 0.84 0.92 0.92 1], y_out=[-1 -1  1  1 -1 -1 -1 -1 -1 -1]}
      mask prompts: edge "Edge Type"; polarity "Output Polarity"; x_in "Input X Positions"; y_in "Input Y Positions"; x_out "Output X Positions"; y_out "Output Y Positions"
      mask help: Output is active for one-cycle after each edge of the specified type (i.e. rising, falling or both).
      mask init: same as ami_fx_sbl_wide/edge_detect
      settings: AttributesFormatString=|
      | rising edges
      | active high
      mask Help: Output is active for one-cycle after each edge of the specified type (i.e. rising, falling, or both).  Latency is zero.
      mask TypeOptions edge: Rising | Falling | Both
      mask TypeOptions polarity: Active High | Active Low
      mask Display:
      | plot(x_in_num,0.5+y_in_num*0.2);
      | plot(x_out_num,0.5+y_out_num*0.2);
  posedge24 : Subsystem  AncestorBlock=casper_library_misc/edge_detect  mask(edge_detect){edge=Rising, polarity=Active High, x_in=[0 0.08 0.08 0.16 0.16 0.24 0.24 0.32 0.32 0.4], y_in=[-1 -1  1  1  1  1  1  1  1  1], x_out=[0.6 0.68 0.68 0.76 0.76 0.84 0.84 0.92 0.92 1], y_out=[-1 -1  1  1 -1 -1 -1 -1 -1 -1]}
      mask prompts: edge "Edge Type"; polarity "Output Polarity"; x_in "Input X Positions"; y_in "Input Y Positions"; x_out "Output X Positions"; y_out "Output Y Positions"
      mask help: Output is active for one-cycle after each edge of the specified type (i.e. rising, falling or both).
      mask init: same as ami_fx_sbl_wide/edge_detect
      settings: AttributesFormatString=|
      | rising edges
      | active high
      mask Help: Output is active for one-cycle after each edge of the specified type (i.e. rising, falling, or both).  Latency is zero.
      mask TypeOptions edge: Rising | Falling | Both
      mask TypeOptions polarity: Active High | Active Low
      mask Display:
      | plot(x_in_num,0.5+y_in_num*0.2);
      | plot(x_out_num,0.5+y_out_num*0.2);
  posedge3 : Subsystem  AncestorBlock=casper_library_misc/edge_detect  mask(edge_detect){edge=Rising, polarity=Active High, x_in=[0 0.08 0.08 0.16 0.16 0.24 0.24 0.32 0.32 0.4], y_in=[-1 -1  1  1  1  1  1  1  1  1], x_out=[0.6 0.68 0.68 0.76 0.76 0.84 0.84 0.92 0.92 1], y_out=[-1 -1  1  1 -1 -1 -1 -1 -1 -1]}
      mask prompts: edge "Edge Type"; polarity "Output Polarity"; x_in "Input X Positions"; y_in "Input Y Positions"; x_out "Output X Positions"; y_out "Output Y Positions"
      mask help: Output is active for one-cycle after each edge of the specified type (i.e. rising, falling or both).
      mask init: same as ami_fx_sbl_wide/edge_detect
      settings: AttributesFormatString=|
      | rising edges
      | active high
      mask Help: Output is active for one-cycle after each edge of the specified type (i.e. rising, falling, or both).  Latency is zero.
      mask TypeOptions edge: Rising | Falling | Both
      mask TypeOptions polarity: Active High | Active Low
      mask Display:
      | plot(x_in_num,0.5+y_in_num*0.2);
      | plot(x_out_num,0.5+y_out_num*0.2);
  pps_count : Subsystem  Tag=xps:sw_reg  mask{io_dir=To Processor, arith_type=Unsigned, bitwidth=32, bin_pt=0, sample_period=1, latency=0}
      link override convert: arith_type=Unsigned  n_bits=32  bin_pt=0
      mask prompts: io_dir "I/O direction"; arith_type "Data Type"; bitwidth "Data bitwidth"; bin_pt "Data binary point"; sample_period "Sample period"
      mask init:
      | gw_name = clear_name(gcb);
      | config.source = str2func('software_register_init');
      | config.toplevel = gcb;
      | xBlock( config, {io_dir, arith_type, bitwidth, bin_pt, ... 
      |     sample_period, gw_name, latency});
      mask TypeOptions io_dir: From Processor | To Processor
      mask TypeOptions arith_type: Unsigned | Signed  (2's comp)
  quantizer_core : xps_library/pcore  Tag=xps:pcore  pcore_path=quantizer_core/quantizer_core.ngc
  rcs : Subsystem  AncestorBlock=casper_library_misc/rcs  mask(rcs){app_src=git, lib_src=git, user_val=429}
      mask prompts: app_src "Application revision info to capture"; lib_src "CASPER libraries revision info to capture"; user_val "User specified value"
      mask help:
      | Embeds revision control information for the user design and libraries.
      | On failure to locate specified revision information, falls back to
      | timestamps (current time for libraries).
      | A user specified value is also stored.
      mask init:
      | rcs_init(gcb, ...
      |     'app_src', app_src, ...
      |     'lib_src', lib_src);
      mask TypeOptions app_src: timestamp | git | svn
      mask TypeOptions lib_src: timestamp | git | svn
  reint : Subsystem
  reint1 : Subsystem
  reorder1 : Subsystem  AncestorBlock=casper_library_reorder/reorder  mask(reorder){n_inputs=1, bram_latency=3, map_latency=3, double_buffer=1, bram_map=on}
      mask prompts: n_inputs "Number of inputs"; bram_latency "BRAM Latency"; map_latency "Map Latency"; double_buffer "Double Buffer"; bram_map "Use BlockRAM for Map"
      mask init:
      | NFFT = 2048;
      | NP = 8;
      | 
      | reorder = zeros(1,NFFT);
      | 
      | part_reorder = [0:NFFT/NP:NFFT-1]
      | 
      | for n = [0:NFFT/NP - 1]
      |     reorder(n*NP+1:(n+1)*NP) = part_reorder+n;
      | end
      | 
      | reorder
      | 
      | map=reorder
      | 
      | 
      | reorder_init(gcb, ...
      |     'map', map, ...
      |     'n_inputs', n_inputs, ...
      |     'bram_latency', bram_latency, ...
      |     'map_latency', map_latency, ...
      |     'double_buffer', double_buffer, ...
      |     'bram_map', bram_map);
      settings: AttributesFormatString=order=2
      mask Help: eval('xlWeb(''http://casper.berkeley.edu/wiki/Reorder'')')
  reorder3 : Subsystem  AncestorBlock=casper_library_reorder/reorder  mask(reorder){n_inputs=1, bram_latency=3, map_latency=3, double_buffer=1, bram_map=on}
      mask prompts: n_inputs "Number of inputs"; bram_latency "BRAM Latency"; map_latency "Map Latency"; double_buffer "Double Buffer"; bram_map "Use BlockRAM for Map"
      mask init: same as ami_fx_sbl_wide/reorder1
      settings: AttributesFormatString=order=2
      mask Help: eval('xlWeb(''http://casper.berkeley.edu/wiki/Reorder'')')
  roach_gpioa6 : xps_library/gpio  Tag=xps:gpio  io_group=ROACH2:gpio  io_dir=in  arith_type=Boolean  bitwidth=1  bin_pt=0  bit_index=6  sample_period=1  use_single_ended=off  use_ddr=off  reg_iob=on  reg_clk_phase=0  termination=None
  roach_gpioa7 : xps_library/gpio  Tag=xps:gpio  io_group=ROACH2:gpio  io_dir=in  arith_type=Boolean  bitwidth=1  bin_pt=0  bit_index=7  sample_period=1  use_single_ended=off  use_ddr=off  reg_iob=on  reg_clk_phase=0  termination=None
  simple_bram_vacc : Subsystem  AncestorBlock=casper_library_accumulators/simple_bram_vacc  mask(simple_bram_vacc){vec_len=2048, arith_type=Signed, n_bits=64, bin_pt=0}
      mask prompts: vec_len "Vector length:"; arith_type "Output type:"; n_bits "Bit width (output):"; bin_pt "Binary point (output):"
      mask help: This simple vector accumulator is based on a shift register. It outputs its previous accumulated vector after a new_acc pulse is received.
      mask init:
      | simple_bram_vacc_init(gcb, ...
      |     'vec_len', vec_len, ...
      |     'arith_type', arith_type, ...
      |     'n_bits', n_bits, ...
      |     'bin_pt', bin_pt);
      mask TypeOptions arith_type: Signed | Unsigned
  simple_bram_vacc1 : Subsystem  AncestorBlock=casper_library_accumulators/simple_bram_vacc  mask(simple_bram_vacc){vec_len=2048, arith_type=Signed, n_bits=64, bin_pt=0}
      mask prompts: vec_len "Vector length:"; arith_type "Output type:"; n_bits "Bit width (output):"; bin_pt "Binary point (output):"
      mask help: This simple vector accumulator is based on a shift register. It outputs its previous accumulated vector after a new_acc pulse is received.
      mask init:
      | simple_bram_vacc_init(gcb, ...
      |     'vec_len', vec_len, ...
      |     'arith_type', arith_type, ...
      |     'n_bits', n_bits, ...
      |     'bin_pt', bin_pt);
      mask TypeOptions arith_type: Signed | Unsigned
  simple_bram_vacc2 : Subsystem  AncestorBlock=casper_library_accumulators/simple_bram_vacc  mask(simple_bram_vacc){vec_len=2048, arith_type=Signed, n_bits=64, bin_pt=0}
      mask prompts: vec_len "Vector length:"; arith_type "Output type:"; n_bits "Bit width (output):"; bin_pt "Binary point (output):"
      mask help: This simple vector accumulator is based on a shift register. It outputs its previous accumulated vector after a new_acc pulse is received.
      mask init:
      | simple_bram_vacc_init(gcb, ...
      |     'vec_len', vec_len, ...
      |     'arith_type', arith_type, ...
      |     'n_bits', n_bits, ...
      |     'bin_pt', bin_pt);
      mask TypeOptions arith_type: Signed | Unsigned
  simple_bram_vacc3 : Subsystem  AncestorBlock=casper_library_accumulators/simple_bram_vacc  mask(simple_bram_vacc){vec_len=2048, arith_type=Signed, n_bits=64, bin_pt=0}
      mask prompts: vec_len "Vector length:"; arith_type "Output type:"; n_bits "Bit width (output):"; bin_pt "Binary point (output):"
      mask help: This simple vector accumulator is based on a shift register. It outputs its previous accumulated vector after a new_acc pulse is received.
      mask init:
      | simple_bram_vacc_init(gcb, ...
      |     'vec_len', vec_len, ...
      |     'arith_type', arith_type, ...
      |     'n_bits', n_bits, ...
      |     'bin_pt', bin_pt);
      mask TypeOptions arith_type: Signed | Unsigned
  snapshot_adc0 : Subsystem  Tag=casper:snapshot  AncestorBlock=casper_library_scopes/snapshot  mask(snapshot){storage=bram, dram_dimm=1, dram_clock=200, nsamples=10, data_width=128, offset=off, circap=off, value=off, use_dsp48=off}
      mask prompts: storage "Storage medium"; dram_dimm "DRAM dimm"; dram_clock "DRAM clock rate"; nsamples "Number of Samples (2^?)"; data_width "Data width"; offset "Start delay support"; circap "Circular capture support"; value "Extra value capture support"; use_dsp48 "Use DSP48s to implement counters"
      mask help:
      | Standard snap block, but with the following optional extras;
      |  1) Optionally delay the fabric trigger by a user-specified number of valids.
      |  2) Capture continuously after a trigger until a stop pulse is received. Data is captured into BRAM continuously, with old data being overwritten until a stop command is received. Then stop capturing when memory is filled. This enables you to get some data before and some data after the stop pulse. Use the 'tr_en_cnt' register to determine where you are in your vector. 'Addr' register's MSb now indicates 'busy capturing'.
      |  3) Optionally capture a value on an input port to a register at the same time as the first data sample.
      |  4) Implement counters using DSP48Es to save resources.
      mask init: same as ami_fx_sbl_wide/corr00
      mask TypeOptions storage: bram | dram
      mask Callback storage: snapshot_callback();
      mask TypeOptions dram_dimm: 1 | 2 | 3 | 4
      mask TypeOptions dram_clock: 200 | 250 | 266 | 300 | 333
      mask TypeOptions data_width: 8 | 16 | 32 | 64 | 128
  snapshot_adc1 : Subsystem  Tag=casper:snapshot  AncestorBlock=casper_library_scopes/snapshot  mask(snapshot){storage=bram, dram_dimm=1, dram_clock=200, nsamples=10, data_width=128, offset=off, circap=off, value=off, use_dsp48=off}
      mask prompts: storage "Storage medium"; dram_dimm "DRAM dimm"; dram_clock "DRAM clock rate"; nsamples "Number of Samples (2^?)"; data_width "Data width"; offset "Start delay support"; circap "Circular capture support"; value "Extra value capture support"; use_dsp48 "Use DSP48s to implement counters"
      mask help:
      | Standard snap block, but with the following optional extras;
      |  1) Optionally delay the fabric trigger by a user-specified number of valids.
      |  2) Capture continuously after a trigger until a stop pulse is received. Data is captured into BRAM continuously, with old data being overwritten until a stop command is received. Then stop capturing when memory is filled. This enables you to get some data before and some data after the stop pulse. Use the 'tr_en_cnt' register to determine where you are in your vector. 'Addr' register's MSb now indicates 'busy capturing'.
      |  3) Optionally capture a value on an input port to a register at the same time as the first data sample.
      |  4) Implement counters using DSP48Es to save resources.
      mask init: same as ami_fx_sbl_wide/corr00
      mask TypeOptions storage: bram | dram
      mask Callback storage: snapshot_callback();
      mask TypeOptions dram_dimm: 1 | 2 | 3 | 4
      mask TypeOptions dram_clock: 200 | 250 | 266 | 300 | 333
      mask TypeOptions data_width: 8 | 16 | 32 | 64 | 128
  snapshot_delay1 : Subsystem  Tag=casper:snapshot  AncestorBlock=casper_library_scopes/snapshot  mask(snapshot){storage=bram, dram_dimm=1, dram_clock=200, nsamples=12, data_width=8, offset=off, circap=off, value=off, use_dsp48=on}
      mask prompts: storage "Storage medium"; dram_dimm "DRAM dimm"; dram_clock "DRAM clock rate"; nsamples "Number of Samples (2^?)"; data_width "Data width"; offset "Start delay support"; circap "Circular capture support"; value "Extra value capture support"; use_dsp48 "Use DSP48s to implement counters"
      mask help:
      | Standard snap block, but with the following optional extras;
      |  1) Optionally delay the fabric trigger by a user-specified number of valids.
      |  2) Capture continuously after a trigger until a stop pulse is received. Data is captured into BRAM continuously, with old data being overwritten until a stop command is received. Then stop capturing when memory is filled. This enables you to get some data before and some data after the stop pulse. Use the 'tr_en_cnt' register to determine where you are in your vector. 'Addr' register's MSb now indicates 'busy capturing'.
      |  3) Optionally capture a value on an input port to a register at the same time as the first data sample.
      |  4) Implement counters using DSP48Es to save resources.
      mask init: same as ami_fx_sbl_wide/corr00
      mask TypeOptions storage: bram | dram
      mask Callback storage: snapshot_callback();
      mask TypeOptions dram_dimm: 1 | 2 | 3 | 4
      mask TypeOptions dram_clock: 200 | 250 | 266 | 300 | 333
      mask TypeOptions data_width: 8 | 16 | 32 | 64 | 128
  snapshot_fd_im1 : Subsystem  Tag=casper:snapshot  AncestorBlock=casper_library_scopes/snapshot  mask(snapshot){storage=bram, dram_dimm=1, dram_clock=200, nsamples=10, data_width=32, offset=off, circap=off, value=off, use_dsp48=on}
      mask prompts: storage "Storage medium"; dram_dimm "DRAM dimm"; dram_clock "DRAM clock rate"; nsamples "Number of Samples (2^?)"; data_width "Data width"; offset "Start delay support"; circap "Circular capture support"; value "Extra value capture support"; use_dsp48 "Use DSP48s to implement counters"
      mask help:
      | Standard snap block, but with the following optional extras;
      |  1) Optionally delay the fabric trigger by a user-specified number of valids.
      |  2) Capture continuously after a trigger until a stop pulse is received. Data is captured into BRAM continuously, with old data being overwritten until a stop command is received. Then stop capturing when memory is filled. This enables you to get some data before and some data after the stop pulse. Use the 'tr_en_cnt' register to determine where you are in your vector. 'Addr' register's MSb now indicates 'busy capturing'.
      |  3) Optionally capture a value on an input port to a register at the same time as the first data sample.
      |  4) Implement counters using DSP48Es to save resources.
      mask init: same as ami_fx_sbl_wide/corr00
      mask TypeOptions storage: bram | dram
      mask Callback storage: snapshot_callback();
      mask TypeOptions dram_dimm: 1 | 2 | 3 | 4
      mask TypeOptions dram_clock: 200 | 250 | 266 | 300 | 333
      mask TypeOptions data_width: 8 | 16 | 32 | 64 | 128
  snapshot_fd_r1 : Subsystem  Tag=casper:snapshot  AncestorBlock=casper_library_scopes/snapshot  mask(snapshot){storage=bram, dram_dimm=1, dram_clock=200, nsamples=10, data_width=32, offset=off, circap=off, value=off, use_dsp48=on}
      mask prompts: storage "Storage medium"; dram_dimm "DRAM dimm"; dram_clock "DRAM clock rate"; nsamples "Number of Samples (2^?)"; data_width "Data width"; offset "Start delay support"; circap "Circular capture support"; value "Extra value capture support"; use_dsp48 "Use DSP48s to implement counters"
      mask help:
      | Standard snap block, but with the following optional extras;
      |  1) Optionally delay the fabric trigger by a user-specified number of valids.
      |  2) Capture continuously after a trigger until a stop pulse is received. Data is captured into BRAM continuously, with old data being overwritten until a stop command is received. Then stop capturing when memory is filled. This enables you to get some data before and some data after the stop pulse. Use the 'tr_en_cnt' register to determine where you are in your vector. 'Addr' register's MSb now indicates 'busy capturing'.
      |  3) Optionally capture a value on an input port to a register at the same time as the first data sample.
      |  4) Implement counters using DSP48Es to save resources.
      mask init: same as ami_fx_sbl_wide/corr00
      mask TypeOptions storage: bram | dram
      mask Callback storage: snapshot_callback();
      mask TypeOptions dram_dimm: 1 | 2 | 3 | 4
      mask TypeOptions dram_clock: 200 | 250 | 266 | 300 | 333
      mask TypeOptions data_width: 8 | 16 | 32 | 64 | 128
  snapshot_fft_i1 : Subsystem  Tag=casper:snapshot  AncestorBlock=casper_library_scopes/snapshot  mask(snapshot){storage=bram, dram_dimm=1, dram_clock=200, nsamples=10, data_width=32, offset=off, circap=off, value=off, use_dsp48=on}
      mask prompts: storage "Storage medium"; dram_dimm "DRAM dimm"; dram_clock "DRAM clock rate"; nsamples "Number of Samples (2^?)"; data_width "Data width"; offset "Start delay support"; circap "Circular capture support"; value "Extra value capture support"; use_dsp48 "Use DSP48s to implement counters"
      mask help:
      | Standard snap block, but with the following optional extras;
      |  1) Optionally delay the fabric trigger by a user-specified number of valids.
      |  2) Capture continuously after a trigger until a stop pulse is received. Data is captured into BRAM continuously, with old data being overwritten until a stop command is received. Then stop capturing when memory is filled. This enables you to get some data before and some data after the stop pulse. Use the 'tr_en_cnt' register to determine where you are in your vector. 'Addr' register's MSb now indicates 'busy capturing'.
      |  3) Optionally capture a value on an input port to a register at the same time as the first data sample.
      |  4) Implement counters using DSP48Es to save resources.
      mask init: same as ami_fx_sbl_wide/corr00
      mask TypeOptions storage: bram | dram
      mask Callback storage: snapshot_callback();
      mask TypeOptions dram_dimm: 1 | 2 | 3 | 4
      mask TypeOptions dram_clock: 200 | 250 | 266 | 300 | 333
      mask TypeOptions data_width: 8 | 16 | 32 | 64 | 128
  snapshot_fft_in1 : Subsystem  Tag=casper:snapshot  AncestorBlock=casper_library_scopes/snapshot  mask(snapshot){storage=bram, dram_dimm=1, dram_clock=200, nsamples=10, data_width=32, offset=off, circap=off, value=off, use_dsp48=on}
      mask prompts: storage "Storage medium"; dram_dimm "DRAM dimm"; dram_clock "DRAM clock rate"; nsamples "Number of Samples (2^?)"; data_width "Data width"; offset "Start delay support"; circap "Circular capture support"; value "Extra value capture support"; use_dsp48 "Use DSP48s to implement counters"
      mask help:
      | Standard snap block, but with the following optional extras;
      |  1) Optionally delay the fabric trigger by a user-specified number of valids.
      |  2) Capture continuously after a trigger until a stop pulse is received. Data is captured into BRAM continuously, with old data being overwritten until a stop command is received. Then stop capturing when memory is filled. This enables you to get some data before and some data after the stop pulse. Use the 'tr_en_cnt' register to determine where you are in your vector. 'Addr' register's MSb now indicates 'busy capturing'.
      |  3) Optionally capture a value on an input port to a register at the same time as the first data sample.
      |  4) Implement counters using DSP48Es to save resources.
      mask init: same as ami_fx_sbl_wide/corr00
      mask TypeOptions storage: bram | dram
      mask Callback storage: snapshot_callback();
      mask TypeOptions dram_dimm: 1 | 2 | 3 | 4
      mask TypeOptions dram_clock: 200 | 250 | 266 | 300 | 333
      mask TypeOptions data_width: 8 | 16 | 32 | 64 | 128
  snapshot_fft_r1 : Subsystem  Tag=casper:snapshot  AncestorBlock=casper_library_scopes/snapshot  mask(snapshot){storage=bram, dram_dimm=1, dram_clock=200, nsamples=10, data_width=32, offset=off, circap=off, value=off, use_dsp48=on}
      mask prompts: storage "Storage medium"; dram_dimm "DRAM dimm"; dram_clock "DRAM clock rate"; nsamples "Number of Samples (2^?)"; data_width "Data width"; offset "Start delay support"; circap "Circular capture support"; value "Extra value capture support"; use_dsp48 "Use DSP48s to implement counters"
      mask help:
      | Standard snap block, but with the following optional extras;
      |  1) Optionally delay the fabric trigger by a user-specified number of valids.
      |  2) Capture continuously after a trigger until a stop pulse is received. Data is captured into BRAM continuously, with old data being overwritten until a stop command is received. Then stop capturing when memory is filled. This enables you to get some data before and some data after the stop pulse. Use the 'tr_en_cnt' register to determine where you are in your vector. 'Addr' register's MSb now indicates 'busy capturing'.
      |  3) Optionally capture a value on an input port to a register at the same time as the first data sample.
      |  4) Implement counters using DSP48Es to save resources.
      mask init: same as ami_fx_sbl_wide/corr00
      mask TypeOptions storage: bram | dram
      mask Callback storage: snapshot_callback();
      mask TypeOptions dram_dimm: 1 | 2 | 3 | 4
      mask TypeOptions dram_clock: 200 | 250 | 266 | 300 | 333
      mask TypeOptions data_width: 8 | 16 | 32 | 64 | 128
  snapshot_fir1 : Subsystem  Tag=casper:snapshot  AncestorBlock=casper_library_scopes/snapshot  mask(snapshot){storage=bram, dram_dimm=1, dram_clock=200, nsamples=10, data_width=32, offset=off, circap=off, value=off, use_dsp48=on}
      mask prompts: storage "Storage medium"; dram_dimm "DRAM dimm"; dram_clock "DRAM clock rate"; nsamples "Number of Samples (2^?)"; data_width "Data width"; offset "Start delay support"; circap "Circular capture support"; value "Extra value capture support"; use_dsp48 "Use DSP48s to implement counters"
      mask help:
      | Standard snap block, but with the following optional extras;
      |  1) Optionally delay the fabric trigger by a user-specified number of valids.
      |  2) Capture continuously after a trigger until a stop pulse is received. Data is captured into BRAM continuously, with old data being overwritten until a stop command is received. Then stop capturing when memory is filled. This enables you to get some data before and some data after the stop pulse. Use the 'tr_en_cnt' register to determine where you are in your vector. 'Addr' register's MSb now indicates 'busy capturing'.
      |  3) Optionally capture a value on an input port to a register at the same time as the first data sample.
      |  4) Implement counters using DSP48Es to save resources.
      mask init: same as ami_fx_sbl_wide/corr00
      mask TypeOptions storage: bram | dram
      mask Callback storage: snapshot_callback();
      mask TypeOptions dram_dimm: 1 | 2 | 3 | 4
      mask TypeOptions dram_clock: 200 | 250 | 266 | 300 | 333
      mask TypeOptions data_width: 8 | 16 | 32 | 64 | 128
  snapshot_pre_vacc : Subsystem  Tag=casper:snapshot  AncestorBlock=casper_library_scopes/snapshot  mask(snapshot){storage=bram, dram_dimm=1, dram_clock=200, nsamples=10, data_width=64, offset=off, circap=off, value=off, use_dsp48=on}
      mask prompts: storage "Storage medium"; dram_dimm "DRAM dimm"; dram_clock "DRAM clock rate"; nsamples "Number of Samples (2^?)"; data_width "Data width"; offset "Start delay support"; circap "Circular capture support"; value "Extra value capture support"; use_dsp48 "Use DSP48s to implement counters"
      mask help:
      | Standard snap block, but with the following optional extras;
      |  1) Optionally delay the fabric trigger by a user-specified number of valids.
      |  2) Capture continuously after a trigger until a stop pulse is received. Data is captured into BRAM continuously, with old data being overwritten until a stop command is received. Then stop capturing when memory is filled. This enables you to get some data before and some data after the stop pulse. Use the 'tr_en_cnt' register to determine where you are in your vector. 'Addr' register's MSb now indicates 'busy capturing'.
      |  3) Optionally capture a value on an input port to a register at the same time as the first data sample.
      |  4) Implement counters using DSP48Es to save resources.
      mask init: same as ami_fx_sbl_wide/corr00
      mask TypeOptions storage: bram | dram
      mask Callback storage: snapshot_callback();
      mask TypeOptions dram_dimm: 1 | 2 | 3 | 4
      mask TypeOptions dram_clock: 200 | 250 | 266 | 300 | 333
      mask TypeOptions data_width: 8 | 16 | 32 | 64 | 128
  sync_gen1 : Subsystem  mask(sync_gen){period_bits=11, acc_bits=24}
      mask prompts: period_bits "sync period (2^?)"; acc_bits "max accumulation length in blocks (2^?)"
      mask help:
      | This block computes the sync period based on system parameters as
      | described in Casper memo.  Detailed descritions of the block's
      | variables can be found in the 'Block Documentation' section of
      | the CASPER wiki.
      mask init:
      | fmtstr = sprintf('sync_period=%d ',2^period_bits);
      | set_param(gcb, 'AttributesFormatString', fmtstr);
      settings: AttributesFormatString=sync_period=2048
      mask Help:
      | SyncPeriod=LCM(reorder_vec)*(acc_num)*(pfb_fir_len)*(fft_size/fft_simult_inputs)
      | 
      | See CASPER sync pulse memo for more details.
  timing : Subsystem  mask{reset_period=1, sync_gen_bits=30}
      mask prompts: reset_period "Master reset time (sync pulses)"; sync_gen_bits "Size of sync generator counter (bits)"
  transpose1 : Subsystem
  transpose2 : Subsystem
  tvg_tr : Subsystem  mask{cnt_bits=8, time_bits=48}
      mask prompts: cnt_bits "Bits in status counters"; time_bits "No LSBs in time to compare"
  ucf : xps_library/ucf  Tag=xps:ucf  ucf_file=user_constraints_sbl_wide.ucf
  unbus0_0 : Subsystem  AncestorBlock=casper_library_flow_control/bus_expand  mask(bus_expand){mode=divisions of equal size, outputNum=16, outputWidth=8, outputBinaryPt=0, outputArithmeticType=0, show_format=off, outputToWorkspace=off, variablePrefix=out, outputToModelAsWell=on}
      mask prompts: outputNum "Number of outputs:"; outputWidth "Output width:"; outputBinaryPt "Output binary point position:"; outputArithmeticType "Output arithmetic type (ufix=0, fix=1, bool=2):"; show_format "Print format string?"; outputToWorkspace "Output to workspace?"; variablePrefix "Variable name prefix:"; outputToModelAsWell "Output to model as well?"
      mask help:
      | Expands a 'bus' made using a bus_create or Xilinx
      | concat block.
      | The input will be divided into the specified number
      | of outputs with the specified arithmetic types.
      | Divisions are made from most significant bit.
      mask init: same as ami_fx_sbl_wide/bus_expand
      settings: AttributesFormatString=16 outputs
      mask TypeOptions mode: divisions of equal size | divisions of arbitrary size
      mask Callback mode: bus_expand_callback();
      mask Callback outputWidth: bus_expand_callback();
      mask Callback outputToWorkspace: bus_expand_callback();
  unbus0_1 : Subsystem  AncestorBlock=casper_library_flow_control/bus_expand  mask(bus_expand){mode=divisions of equal size, outputNum=16, outputWidth=8, outputBinaryPt=0, outputArithmeticType=0, show_format=off, outputToWorkspace=off, variablePrefix=out, outputToModelAsWell=on}
      mask prompts: outputNum "Number of outputs:"; outputWidth "Output width:"; outputBinaryPt "Output binary point position:"; outputArithmeticType "Output arithmetic type (ufix=0, fix=1, bool=2):"; show_format "Print format string?"; outputToWorkspace "Output to workspace?"; variablePrefix "Variable name prefix:"; outputToModelAsWell "Output to model as well?"
      mask help:
      | Expands a 'bus' made using a bus_create or Xilinx
      | concat block.
      | The input will be divided into the specified number
      | of outputs with the specified arithmetic types.
      | Divisions are made from most significant bit.
      mask init: same as ami_fx_sbl_wide/bus_expand
      settings: AttributesFormatString=16 outputs
      mask TypeOptions mode: divisions of equal size | divisions of arbitrary size
      mask Callback mode: bus_expand_callback();
      mask Callback outputWidth: bus_expand_callback();
      mask Callback outputToWorkspace: bus_expand_callback();
  wires:
  pipeline49/1(q) -> fd_local_time/2(sync), Delay20/1
  fine_del0/1 -> pipeline79/1(d)
  Constant10/1 -> [quant_or0]
  [mrst] -> cd_local_time/1(reset)
  [sync] -> cd_local_time/2(sync)
  cd_local_time/1(time) -> [cd_local_time]
  Constant33/1 -> ld_time_msw0/1(sim_1)
  Constant29/1 -> ld_time_lsw0/1(sim_1)
  ld_time_msw0/1(in_reg) -> Slice73/1, Slice7/1
  Slice73/1 -> Concat9/1
  ld_time_lsw0/1(in_reg) -> Concat9/2
  fstatus0/1(sim_reg_out) -> Terminator9/1
  Constant18/1 -> control/1(sim_1)
  control/1(in_reg) -> Delay6/1
  Delay6/1 -> Slice78/1, man_sync1/1, arm1/1, arm2/1, arm8/1, arm10/1, arm6/1, arm13/1, arm7/1, arm5/1, arm4/1, arm3/1, arm11/1, arm9/1, arm12/1
  Slice78/1 -> [sys_rst]
  man_sync1/1 -> posedge1/1(in)
  posedge1/1(out) -> [man_sync]
  arm1/1 -> posedge24/1(in)
  posedge24/1(out) -> [arm]
  arm2/1 -> posedge23/1(in)
  posedge23/1(out) -> [clr_status]
  mcount_msw/1(sim_reg_out) -> Terminator12/1
  mcount_lsw/1(sim_reg_out) -> Terminator13/1
  Slice/1 -> mcount_lsw/1(reg_out)
  Slice1/1 -> mcount_msw/1(reg_out)
  fstatus1/1(sim_reg_out) -> Terminator2/1
  Constant32/1 -> coarse_delay0/1(sim_1)
  Constant8/1 -> a0_fd0/1(sim_1)
  Constant4/1 -> a1_fd0/1(sim_1)
  a0_fd0/1(in_reg) -> Slice3/1, Slice2/1
  Slice4/1 -> Concat22/4
  Slice5/1 -> Concat22/5
  cd_tr0/1(arm_count) -> Terminator14/1
  edge_detect1/1(out) -> [adc_sync0]
  [mrst] -> fd_local_time/1(reset)
  fd_local_time/1(time) -> tvg_tr/4(current_time), Delay24/1
  calc_adc_sum_sq/1(sum_sq) -> Delay8/1
  [adc0] -> pipeline47/1(d)
  adc_sum_sq0/1(sim_reg_out) -> Terminator/1
  [adc1] -> pipeline48/1(d)
  calc_adc_sum_sq1/1(sum_sq) -> Delay12/1
  adc_sum_sq1/1(sim_reg_out) -> Terminator25/1
  arm3/1 -> posedge2/1(in)
  posedge2/1(out) -> [tvg_en]
  arm4/1 -> [ct_tvg]
  arm5/1 -> [packetiser_tvg]
  arm6/1 -> [fd_fs_tvg]
  [clr_status] -> Subsystem7/1(clr)
  Constant3/1 -> Subsystem7/2(xuai_ldn)
  Constant5/1 -> Subsystem7/3(xaui_of)
  Constant7/1 -> Subsystem7/4(ct_err)
  [adc_or0] -> Subsystem7/5(adc_or)
  [fft_or0] -> Subsystem7/6(fft_or)
  [quant_or0] -> Subsystem7/7(quant_or)
  arm7/1 -> [adc_tvg]
  coarse_delay0/1(in_reg) -> Slice38/1
  Slice2/1 -> Concat22/1
  Slice3/1 -> Concat22/2
  [cd_val1] -> Slice22/1, Slice20/1, Slice23/1, Slice24/1, Slice21/1
  Slice88/1 -> fine_del0/4
  Slice69/1 -> fine_del0/5
  Slice57/1 -> fine_del0/3
  Slice58/1 -> fine_del0/6
  Slice56/1 -> fine_del0/7
  delay_gen0/4(phase_out) -> Terminator35/1
  delay_gen0/5(slope_out) -> Terminator36/1
  delay_gen0/7(idx_d0) -> Terminator37/1
  delay_gen0/8(d1) -> Terminator38/1
  delay_gen0/9(idx_d1) -> Terminator39/1
  delay_gen1/9(idx_d1) -> Terminator44/1
  delay_gen1/8(d1) -> Terminator43/1
  delay_gen1/7(idx_d0) -> Terminator42/1
  delay_gen1/4(phase_out) -> Terminator40/1
  delay_gen1/5(slope_out) -> Terminator41/1
  delay_gen1/6(d0) -> unbus0_1/1(bus_in)
  arm8/1 -> Delay100/1(d)
  arm9/1 -> Delay2/1(d)
  Delay100/1(q) -> [gbe_enable]
  Delay2/1(q) -> [gbe_rst]
  arm10/1 -> [fancy_en]
  [cd_val0] -> Slice16/1, Slice19/1, Slice18/1, Slice15/1, Slice17/1
  [cd_en0] -> delay_gen0/2(en)
  Slice16/1 -> delay_gen0/3(phase)
  Slice19/1 -> delay_gen0/4(d/dt_phase)
  Constant17/1 -> delay_gen0/8(din1)
  Slice18/1 -> Concat4/1
  Slice17/1 -> Concat4/2
  Concat4/1 -> delay_gen0/5(delay)
  Slice15/1 -> delay_gen0/6(d/dt_delay)
  Constant19/1 -> delay_gen0/9(invert_slope)
  [cd_en1] -> delay_gen1/2(en)
  Slice21/1 -> delay_gen1/3(phase)
  Slice24/1 -> delay_gen1/4(d/dt_phase)
  Constant21/1 -> delay_gen1/8(din1)
  Slice23/1 -> Concat5/1
  Slice22/1 -> Concat5/2
  Concat5/1 -> delay_gen1/5(delay)
  Slice20/1 -> delay_gen1/6(d/dt_delay)
  Constant22/1 -> delay_gen1/9(invert_slope)
  adc5g_0/17(sync_out) -> pipeline12/1(d)
  [sync_raw0] -> edge_detect1/1(in)
  [sync_val0] -> Subsystem7/8(sync_val)
  arm11/1 -> [adc_protect_disable]
  [mrst] -> edge_detect/1(in)
  edge_detect/1(out) -> Delay/1
  [mrst] -> cd_tr0/1(rst)
  Logical11/1 -> cd_tr0/3(arm)
  [cd_local_time] -> cd_tr0/4(current_time)
  [mrst] -> fd_tr0/1(rst)
  Logical12/1 -> pipeline108/1(d)
  [fd_local_time] -> fd_tr0/4(current_time)
  Slice38/1 -> AddSub/1
  [sync_val0] -> AddSub/2
  AddSub/1 -> Concat22/3
  Constant/1 -> [sync_val0]
  Delay8/1 -> adc_sum_sq0/1(reg_out)
  Delay12/1 -> adc_sum_sq1/1(reg_out)
  [cd_local_time] -> pipeline75/1(d)
  Delay/1 -> [load_now]
  Slice7/1 -> [arm0]
  [load_now] -> cd_tr0/2(load_now), Logical11/1
  [arm0] -> Logical11/2
  [arm0] -> Logical12/2
  [load_now] -> Logical12/1, pipeline107/1(d)
  cd_tr0/2(ld_count) -> Terminator15/1
  cd_tr0/3(value) -> [cd_val0]
  cd_tr0/4(enable) -> [cd_en0]
  Concat9/1 -> [ld_time0]
  [ld_time0] -> cd_tr0/5(load_time)
  Concat22/1 -> [ld_val0]
  fd_tr0/1(arm_count) -> Convert4/1
  fd_tr0/2(ld_count) -> Convert5/1
  fd_tr0/3(value) -> Slice57/1, Slice56/1, Slice58/1, Slice69/1, Slice88/1
  [ld_val0] -> cd_tr0/6(load_value)
  [ld_time0] -> fd_tr0/5(load_time)
  [ld_val0] -> fd_tr0/6(load_value)
  a1_fd0/1(in_reg) -> Slice4/1, Slice5/1
  cd_tr1/1(arm_count) -> Terminator16/1
  [mrst] -> cd_tr1/1(rst)
  Logical19/1 -> cd_tr1/3(arm)
  [cd_local_time] -> cd_tr1/4(current_time)
  [load_now] -> Logical19/1, cd_tr1/2(load_now)
  [arm1] -> Logical19/2
  cd_tr1/2(ld_count) -> Terminator18/1
  cd_tr1/3(value) -> [cd_val1]
  cd_tr1/4(enable) -> [cd_en1]
  [ld_time1] -> cd_tr1/5(load_time)
  [ld_val1] -> cd_tr1/6(load_value)
  bus_create/1(bus_out) -> fd_tr0/7(din)
  fd_tr0/5(dout) -> bus_expand1/1(bus_in)
  Slice12/1 -> fine_del1/4
  Slice11/1 -> fine_del1/5
  Slice9/1 -> fine_del1/3
  Slice10/1 -> fine_del1/6
  Slice8/1 -> fine_del1/7
  [mrst] -> fd_tr1/1(rst)
  Logical13/1 -> pipeline110/1(d)
  [fd_local_time] -> fd_tr1/4(current_time)
  [arm1] -> Logical13/2
  [load_now] -> pipeline109/1(d), Logical13/1
  fd_tr1/1(arm_count) -> Convert6/1
  fd_tr1/2(ld_count) -> Convert7/1
  fd_tr1/3(value) -> Slice12/1, Slice11/1, Slice10/1, Slice8/1, Slice9/1
  [ld_time1] -> fd_tr1/5(load_time)
  [ld_val1] -> fd_tr1/6(load_value)
  bus_create1/1(bus_out) -> fd_tr1/7(din)
  fd_tr1/5(dout) -> bus_expand3/1(bus_in)
  bus_expand3/1(msb_out2) -> fine_del1/1
  fd_tr0/4(enable) -> fine_del0/2
  fd_tr1/4(enable) -> fine_del1/2
  [mrst] -> gpio_tr/1(rst)
  Logical15/1 -> gpio_tr/3(arm)
  [cd_local_time] -> gpio_tr/4(current_time)
  [load_now] -> gpio_tr/2(load_now), Logical15/1
  [arm0] -> Logical15/2
  [ld_time0] -> gpio_tr/5(load_time)
  Constant34/1 -> gpio_tr/6(load_value)
  [timing_pps] -> gpio_tr/7(din)
  gpio_tr/5(dout) -> Delay28/1
  gpio_tr/1(arm_count) -> Terminator19/1
  gpio_tr/2(ld_count) -> Terminator21/1
  [mrst] -> tvg_tr/1(rst)
  Logical20/1 -> tvg_tr/3(arm)
  [arm0] -> Logical20/2
  [load_now] -> tvg_tr/2(load_now), Logical20/1
  [ld_time0] -> tvg_tr/5(load_time)
  Constant35/1 -> tvg_tr/6(load_value)
  Constant14/1 -> tvg_tr/7(din)
  tvg_tr/5(dout) -> Terminator23/1
  tvg_tr/1(arm_count) -> Terminator26/1
  tvg_tr/2(ld_count) -> Terminator27/1
  tvg_tr/3(value) -> Terminator29/1
  tvg_tr/4(enable) -> [tvg_tr_en]
  [fd_fs_tvg] -> Register2/1
  Delay24/1 -> [fd_local_time]
  Delay25/1 -> bus_create1/1(in1)
  Logical7/1 -> pipeline9/1(d)
  [sync] -> pipeline6/1(d)
  Logical4/1 -> pipeline4/1(d)
  [pps] -> pipeline5/1(d)
  [mrst] -> pipeline7/1(d)
  [fancy_en] -> pipeline8/1(d)
  Constant44/1 -> Logical4/1
  Constant45/1 -> Logical4/2
  [adc_or1] -> Logical16/1
  [fft_or1] -> Logical16/2
  [adc_or0] -> Logical17/1
  [fft_or0] -> Logical17/2
  Logical17/1 -> pipeline1/1(d)
  Logical16/1 -> pipeline/1(d)
  Constant50/1 -> pipeline3/1(d)
  Constant51/1 -> pipeline2/1(d)
  Constant42/1 -> Logical7/2
  Constant39/1 -> Logical7/1
  [sync] -> Concat10/1
  [data_adc0] -> Concat10/2
  Concat10/1 -> cd_tr0/7(din)
  cd_tr0/5(dout) -> bus_expand5/1(bus_in)
  bus_expand5/1(msb_out2) -> delay_gen0/1(sync_in)
  bus_expand5/2(lsb_out1) -> delay_gen0/7(din0)
  gpio_tr/3(value) -> Terminator28/1
  gpio_tr/4(enable) -> Register4/2
  [tvg_en] -> Register2/2
  [clk_bad] -> Subsystem7/10(clk_bad)
  Constant27/1 -> Subsystem7/9(adc_disable)
  [clr_status] -> Subsystem1/1(clr)
  Constant20/1 -> Subsystem1/2(xuai_ldn)
  Constant26/1 -> Subsystem1/3(xaui_of)
  Constant31/1 -> Subsystem1/4(ct_err)
  [fft_or1] -> Subsystem1/6(fft_or)
  [quant_or1] -> Subsystem1/7(quant_or)
  [sync_val0] -> Subsystem1/8(sync_val)
  [clk_bad] -> Subsystem1/10(clk_bad)
  [arm0] -> edge_detect2/1(in)
  Constant38/1 -> Register4/1
  Register4/1 -> ?
  edge_detect2/1(out) -> Register4/3
  Delay28/1 -> ?
  Constant48/1 -> Logical7/3
  Constant49/1 -> Logical7/4
  [clk_bad] -> Logical7/5
  delay_tr_status0/1(sim_reg_out) -> Terminator17/1
  Convert4/1 -> Concat13/1
  Concat13/1 -> pipeline106/1(d)
  Convert5/1 -> Concat13/2
  delay_tr_status1/1(sim_reg_out) -> Terminator6/1
  Convert6/1 -> Concat14/1
  Concat14/1 -> pipeline105/1(d)
  Convert7/1 -> Concat14/2
  Constant23/1 -> Subsystem7/11(dram_bad)
  Constant43/1 -> Logical7/7
  Constant1/1 -> Logical7/6
  Subsystem7/1(status) -> fstatus0/1(reg_out)
  arm12/1 -> posedge3/1(in)
  posedge3/1(out) -> [clr_adc_bad]
  Constant13/1 -> ld_time_msw1/1(sim_1)
  Constant6/1 -> ld_time_lsw1/1(sim_1)
  ld_time_msw1/1(in_reg) -> Slice32/1, Slice37/1
  Slice37/1 -> Concat2/1
  ld_time_lsw1/1(in_reg) -> Concat2/2
  Constant12/1 -> coarse_delay1/1(sim_1)
  Constant16/1 -> a0_fd1/1(sim_1)
  Constant15/1 -> a1_fd1/1(sim_1)
  a0_fd1/1(in_reg) -> Slice13/1, Slice25/1
  Slice28/1 -> Concat1/4
  Slice31/1 -> Concat1/5
  coarse_delay1/1(in_reg) -> Slice27/1
  Slice13/1 -> Concat1/1
  Slice25/1 -> Concat1/2
  Slice27/1 -> AddSub1/1
  [sync_val0] -> AddSub1/2
  AddSub1/1 -> Concat1/3
  Slice32/1 -> [arm1]
  Concat2/1 -> [ld_time1]
  Concat1/1 -> [ld_val1]
  a1_fd1/1(in_reg) -> Slice31/1, Slice28/1
  Subsystem1/1(status) -> fstatus1/1(reg_out)
  [adc_or1] -> Subsystem1/5(adc_or)
  notused/1 -> [adc_or0], [adc_or1]
  adc5g_1/17(sync_out) -> pipeline10/1(d)
  unbus0_0/1(msb_out16) -> delay_0/4
  unbus0_0/2(out15) -> delay_0/5
  unbus0_0/3(out14) -> delay_0/6
  unbus0_0/4(out13) -> delay_0/7
  unbus0_0/5(out12) -> delay_0/8
  unbus0_0/6(out11) -> delay_0/9
  unbus0_0/7(out10) -> delay_0/10
  unbus0_0/8(out9) -> delay_0/11
  unbus0_0/9(out8) -> delay_0/12
  unbus0_0/10(out7) -> delay_0/13
  unbus0_0/11(out6) -> delay_0/14
  unbus0_0/12(out5) -> delay_0/15
  unbus0_0/13(out4) -> delay_0/16
  unbus0_0/14(out3) -> delay_0/17
  unbus0_0/15(out2) -> delay_0/18
  unbus0_0/16(lsb_out1) -> delay_0/19
  delay_gen0/1(sync_out) -> delay_0/1
  delay_gen0/2(en_out) -> delay_0/3
  delay_gen0/3(cd_o) -> delay_0/2
  delay_gen0/6(d0) -> unbus0_0/1(bus_in)
  unbus0_1/1(msb_out16) -> delay_1/4
  unbus0_1/2(out15) -> delay_1/5
  unbus0_1/3(out14) -> delay_1/6
  unbus0_1/4(out13) -> delay_1/7
  unbus0_1/5(out12) -> delay_1/8
  unbus0_1/6(out11) -> delay_1/9
  unbus0_1/7(out10) -> delay_1/10
  unbus0_1/8(out9) -> delay_1/11
  unbus0_1/9(out8) -> delay_1/12
  unbus0_1/10(out7) -> delay_1/13
  unbus0_1/11(out6) -> delay_1/14
  unbus0_1/12(out5) -> delay_1/15
  unbus0_1/13(out4) -> delay_1/16
  unbus0_1/14(out3) -> delay_1/17
  unbus0_1/15(out2) -> delay_1/18
  unbus0_1/16(lsb_out1) -> delay_1/19
  delay_gen1/1(sync_out) -> delay_1/1
  delay_gen1/2(en_out) -> delay_1/3
  delay_gen1/3(cd_o) -> delay_1/2
  pipeline50/1(q) -> bus_create4/1(in1)
  pipeline51/1(q) -> bus_create4/2(in2)
  pipeline52/1(q) -> bus_create4/3(in3)
  pipeline53/1(q) -> bus_create4/4(in4)
  pipeline54/1(q) -> bus_create4/5(in5)
  pipeline55/1(q) -> bus_create4/6(in6)
  pipeline56/1(q) -> bus_create4/7(in7)
  pipeline57/1(q) -> bus_create4/8(in8)
  bus_create4/1(bus_out) -> Delay22/1
  pipeline59/1(q) -> Delay25/1
  pipeline60/1(q) -> bus_create5/1(in1)
  pipeline61/1(q) -> bus_create5/2(in2)
  pipeline62/1(q) -> bus_create5/3(in3)
  pipeline63/1(q) -> bus_create5/4(in4)
  pipeline64/1(q) -> bus_create5/5(in5)
  pipeline65/1(q) -> bus_create5/6(in6)
  pipeline66/1(q) -> bus_create5/7(in7)
  pipeline67/1(q) -> bus_create5/8(in8)
  bus_create5/1(bus_out) -> Delay26/1
  Delay26/1 -> bus_create1/2(in2)
  bus_expand1/1(msb_out2) -> fine_del0/1
  bus_expand1/2(lsb_out1) -> fine_del0/8
  bus_expand3/2(lsb_out1) -> fine_del1/8
  pipeline78/1(q) -> [quant0_data]
  fine_del1/2 -> Slice30/1, pipeline81/1(d)
  Delay20/1 -> bus_create/1(in1)
  Delay22/1 -> bus_create/2(in2)
  Constant11/1 -> [quant_or1]
  pipeline81/1(q) -> [quant1_data]
  Constant47/1 -> Subsystem1/9(adc_disable)
  [quant0_sync] -> ct_tvg2/2(sync_in)
  [quant0_data] -> ct_tvg2/3(din)
  [ct_tvg] -> Register/1
  [tvg_en] -> Register/2
  Register/1 -> ct_tvg2/1(enable)
  [quant1_sync] -> ct_tvg1/2(sync_in)
  [quant1_data] -> ct_tvg1/3(din)
  [ct_tvg] -> Register6/1
  [tvg_en] -> Register6/2
  Register6/1 -> ct_tvg1/1(enable)
  Reinterpret/1 -> Convert/1
  Convert/1 -> pipeline82/1(d)
  Reinterpret1/1 -> Convert1/1
  Reinterpret2/1 -> Convert2/1
  Convert2/1 -> pipeline84/1(d)
  Convert1/1 -> pipeline83/1(d)
  simple_bram_vacc/1(dout) -> pipeline24/1(d)
  simple_bram_vacc/2(valid) -> edge_detect3/1(in), pipeline23/1(d)
  edge_detect3/1(out) -> corr00/3(trig)
  simple_bram_vacc1/1(dout) -> pipeline22/1(d)
  simple_bram_vacc1/2(valid) -> edge_detect4/1(in), pipeline21/1(d)
  edge_detect4/1(out) -> corr11/3(trig)
  simple_bram_vacc2/2(valid) -> edge_detect5/1(in), pipeline19/1(d)
  edge_detect5/1(out) -> corr01_r/3(trig)
  simple_bram_vacc2/1(dout) -> pipeline20/1(d)
  [reorder_data1] -> pipeline33/1(d)
  [reorder0_sync] -> pipeline31/1(d)
  [reorder_data0] -> pipeline32/1(d)
  Constant24/1 -> Subsystem1/11(dram_bad)
  bus_expand/3(out2) -> Logical1/3
  bus_expand/2(out3) -> Logical1/2
  bus_expand/4(lsb_out1) -> Logical1/4
  bus_expand/1(msb_out4) -> Logical1/1
  pipeline68/1(q) -> bus_expand/1(bus_in)
  Logical1/1 -> Convert8/1
  bus_expand2/3(out2) -> Logical2/3
  bus_expand2/2(out3) -> Logical2/2
  bus_expand2/4(lsb_out1) -> Logical2/4
  bus_expand2/1(msb_out4) -> Logical2/1
  pipeline58/1(q) -> bus_expand2/1(bus_in)
  Logical2/1 -> Convert3/1
  Convert3/1 -> [fft_or0]
  Convert8/1 -> [fft_or1]
  pipeline/1(q) -> leds/10(or1)
  pipeline1/1(q) -> leds/9(or0)
  pipeline2/1(q) -> leds/8(adc_en1)
  pipeline3/1(q) -> leds/7(adc_en0)
  pipeline4/1(q) -> leds/6(comms)
  pipeline5/1(q) -> leds/5(pps)
  pipeline6/1(q) -> leds/4(sync_led)
  pipeline7/1(q) -> leds/3(rst)
  pipeline8/1(q) -> leds/2(fancy_en)
  pipeline9/1(q) -> leds/1(warning)
  pipeline10/1(q) -> [sync_raw1]
  bus_create3/1(bus_out) -> pipeline11/1(d)
  pipeline12/1(q) -> [sync_raw0]
  bus_create2/1(bus_out) -> pipeline13/1(d)
  pipeline19/1(q) -> corr01_r/2(we)
  pipeline20/1(q) -> corr01_r/1(din)
  pipeline21/1(q) -> corr11/2(we)
  pipeline22/1(q) -> corr11/1(din)
  pipeline23/1(q) -> corr00/2(we)
  pipeline24/1(q) -> corr00/1(din)
  pipeline25/1(q) -> simple_bram_vacc/1(new_acc)
  pipeline26/1(q) -> simple_bram_vacc/2(din)
  pipeline27/1(q) -> simple_bram_vacc1/1(new_acc)
  pipeline28/1(q) -> simple_bram_vacc1/2(din)
  pipeline29/1(q) -> simple_bram_vacc2/1(new_acc)
  pipeline30/1(q) -> simple_bram_vacc2/2(din)
  Constant25/1 -> [ct_err0]
  Constant52/1 -> [ct_err1]
  Constant53/1 -> reorder1/2(en)
  ct_tvg1/2(dout) -> reorder1/3(din0)
  ct_tvg1/1(sync_out) -> reorder1/1(sync)
  reorder1/1(sync_out) -> transpose1/1(sync)
  reorder1/3(dout0) -> transpose1/2(din)
  Constant54/1 -> reorder3/2(en)
  ct_tvg2/2(dout) -> reorder3/3(din0)
  ct_tvg2/1(sync_out) -> reorder3/1(sync)
  reorder3/1(sync_out) -> transpose2/1(sync)
  reorder3/3(dout0) -> transpose2/2(din)
  pipeline34/1(q) -> addtree1/1(sync)
  pipeline35/1(q) -> addtree1/2(din00)
  pipeline36/1(q) -> addtree1/3(din11)
  pipeline37/1(q) -> addtree1/4(din01)
  Counter1/1 -> Register19/1
  Register19/1 -> pipeline40/1(d), Relational/1, Relational1/1
  clk_frequency/1(sim_reg_out) -> Terminator10/1
  pps_count/1(sim_reg_out) -> Terminator11/1
  [mrst] -> pipeline43/1(d)
  [armed] -> pipeline42/1(d)
  Counter3/1 -> Concat21/2
  Concat21/1 -> pipeline39/1(d)
  Constant36/1 -> Relational/2
  Constant37/1 -> Relational1/2
  Relational/1 -> Logical21/1
  Relational1/1 -> Logical21/2
  Logical21/1 -> pipeline41/1(d)
  pipeline42/1(q) -> Concat21/1
  pipeline43/1(q) -> Counter3/1
  [pps] -> pipeline76/1(d), pipeline38/1(d), pipeline77/1(d)
  pipeline39/1(q) -> pps_count/1(reg_out)
  pipeline40/1(q) -> clk_frequency/1(reg_out)
  pipeline41/1(q) -> [clk_bad]
  [adc0] -> pipeline45/1(d)
  pipeline45/1(q) -> snapshot_adc0/1(din)
  [adc_sync0] -> pipeline15/1(d)
  timing/2(sync) -> [sync]
  Logical3/1 -> timing/4(pps_in), [pps]
  Concat/1 -> timing/2(data_in)
  timing/1(armed) -> Logical14/2, [armed]
  Logical14/1 -> [mrst]
  [sys_rst] -> Logical14/1
  [man_sync] -> pipeline17/1(d)
  [arm] -> timing/1(arm)
  Constant2/1 -> timing/3(sync_period)
  [adc0] -> pipeline14/1(d)
  [adc1] -> pipeline16/1(d)
  [adc_sync0] -> pipeline18/1(d)
  timing/3(data_out) -> bus_expand6/1(bus_in)
  bus_expand6/3(lsb_out1) -> [data_adc1]
  bus_expand6/2(out2) -> [data_adc0]
  bus_expand6/1(msb_out3) -> [timing_pps]
  pipeline15/1(q) -> Logical3/2
  pipeline17/1(q) -> Logical3/1
  pipeline16/1(q) -> Concat/3
  pipeline14/1(q) -> Concat/2
  pipeline18/1(q) -> Concat/1
  pipeline47/1(q) -> calc_adc_sum_sq/1(In1)
  pipeline48/1(q) -> calc_adc_sum_sq1/1(In1)
  Subsystem2/1(sync_out) -> fir_0/1
  Subsystem2/14(Out13) -> fir_0/14
  Subsystem2/5(Out4) -> fir_0/5
  Subsystem2/4(Out3) -> fir_0/4
  Subsystem2/10(Out9) -> fir_0/10
  Subsystem2/7(Out6) -> fir_0/7
  Subsystem2/3(Out2) -> fir_0/3
  Subsystem2/2(Out1) -> fir_0/2
  Subsystem2/13(Out12) -> fir_0/13
  Subsystem2/12(Out11) -> fir_0/12
  Subsystem2/17(Out16) -> fir_0/17
  Subsystem2/15(Out14) -> fir_0/15
  Subsystem2/16(Out15) -> fir_0/16
  Subsystem2/6(Out5) -> fir_0/6
  Subsystem2/8(Out7) -> fir_0/8
  Subsystem2/9(Out8) -> fir_0/9
  Subsystem2/11(Out10) -> fir_0/11
  Subsystem3/1(sync_out) -> fir_1/1
  Subsystem3/2(Out1) -> fir_1/2
  Subsystem3/3(Out2) -> fir_1/3
  Subsystem3/4(Out3) -> fir_1/4
  Subsystem3/5(Out4) -> fir_1/5
  Subsystem3/6(Out5) -> fir_1/6
  Subsystem3/7(Out6) -> fir_1/7
  Subsystem3/8(Out7) -> fir_1/8
  Subsystem3/9(Out8) -> fir_1/9
  Subsystem3/10(Out9) -> fir_1/10
  Subsystem3/11(Out10) -> fir_1/11
  Subsystem3/12(Out11) -> fir_1/12
  Subsystem3/13(Out12) -> fir_1/13
  Subsystem3/14(Out13) -> fir_1/14
  Subsystem3/15(Out14) -> fir_1/15
  Subsystem3/16(Out15) -> fir_1/16
  Subsystem3/17(Out16) -> fir_1/17
  Constant40/1 -> fft_shift0/1(sim_1)
  fft_shift0/1(in_reg) -> pipeline74/1(d)
  Slice6/1 -> fft_core0/1
  a0p0_1st_shift/1(sync_out) -> fft_core0/2
  a0p0_1st_shift/2(dout1) -> fft_core0/3
  a0p0_1st_shift/3(dout2) -> fft_core0/4
  a0p0_1st_shift/4(dout3) -> fft_core0/5
  a0p0_1st_shift/5(dout4) -> fft_core0/6
  a0p0_1st_shift/6(dout5) -> fft_core0/7
  a0p0_1st_shift/7(dout6) -> fft_core0/8
  a0p0_1st_shift/8(dout7) -> fft_core0/9
  a0p0_1st_shift/9(dout8) -> fft_core0/10
  a0p0_1st_shift/10(dout9) -> fft_core0/11
  a0p0_1st_shift/11(dout10) -> fft_core0/12
  a0p0_1st_shift/12(dout11) -> fft_core0/13
  a0p0_1st_shift/13(dout12) -> fft_core0/14
  a0p0_1st_shift/14(dout13) -> fft_core0/15
  a0p0_1st_shift/15(dout14) -> fft_core0/16
  a0p0_1st_shift/16(dout15) -> fft_core0/17
  a0p0_1st_shift/17(dout16) -> fft_core0/18
  fir_0/2 -> Subsystem4/2(In1)
  fir_0/3 -> Subsystem4/3(In2)
  fir_0/4 -> Subsystem4/4(In3)
  fir_0/15 -> Subsystem4/15(In14)
  fir_0/11 -> Subsystem4/11(In10)
  fir_0/12 -> Subsystem4/12(In11)
  fir_0/5 -> Subsystem4/5(In4)
  fir_0/8 -> Subsystem4/8(In7)
  fir_0/9 -> Subsystem4/9(In8)
  fir_0/10 -> Subsystem4/10(In9)
  fir_0/16 -> Subsystem4/16(In15)
  fir_0/17 -> Subsystem4/17(In16)
  fir_0/13 -> Subsystem4/13(In12)
  fir_0/14 -> Subsystem4/14(In13)
  fir_0/6 -> Subsystem4/6(In5)
  fir_0/7 -> Subsystem4/7(In6)
  fir_0/1 -> Subsystem4/1(sync)
  Subsystem4/6(Out5) -> a0p0_1st_shift/6(din5)
  Subsystem4/9(Out8) -> a0p0_1st_shift/9(din8)
  Subsystem4/14(Out13) -> a0p0_1st_shift/14(din13)
  Subsystem4/16(Out15) -> a0p0_1st_shift/16(din15)
  Subsystem4/12(Out11) -> a0p0_1st_shift/12(din11)
  Subsystem4/2(Out1) -> a0p0_1st_shift/2(din1)
  Subsystem4/17(Out16) -> a0p0_1st_shift/17(din16)
  Subsystem4/4(Out3) -> a0p0_1st_shift/4(din3)
  Subsystem4/10(Out9) -> a0p0_1st_shift/10(din9)
  Subsystem4/7(Out6) -> a0p0_1st_shift/7(din6)
  Subsystem4/5(Out4) -> a0p0_1st_shift/5(din4)
  Subsystem4/13(Out12) -> a0p0_1st_shift/13(din12)
  Subsystem4/8(Out7) -> a0p0_1st_shift/8(din7)
  Subsystem4/1(sync_out) -> a0p0_1st_shift/1(sync_in)
  Subsystem4/3(Out2) -> a0p0_1st_shift/3(din2)
  Subsystem4/15(Out14) -> a0p0_1st_shift/15(din14)
  Subsystem4/11(Out10) -> a0p0_1st_shift/11(din10)
  Constant9/1 -> fft_shift1/1(sim_1)
  fft_shift1/1(in_reg) -> pipeline73/1(d)
  Slice14/1 -> fft_core1/1
  a0p0_1st_shift1/1(sync_out) -> fft_core1/2
  a0p0_1st_shift1/2(dout1) -> pipeline95/1(d), fft_core1/3
  a0p0_1st_shift1/3(dout2) -> fft_core1/4
  a0p0_1st_shift1/4(dout3) -> fft_core1/5
  a0p0_1st_shift1/5(dout4) -> fft_core1/6
  a0p0_1st_shift1/6(dout5) -> fft_core1/7
  a0p0_1st_shift1/7(dout6) -> fft_core1/8
  a0p0_1st_shift1/8(dout7) -> fft_core1/9
  a0p0_1st_shift1/9(dout8) -> fft_core1/10
  a0p0_1st_shift1/10(dout9) -> fft_core1/11
  a0p0_1st_shift1/11(dout10) -> fft_core1/12
  a0p0_1st_shift1/12(dout11) -> fft_core1/13
  a0p0_1st_shift1/13(dout12) -> fft_core1/14
  a0p0_1st_shift1/14(dout13) -> fft_core1/15
  a0p0_1st_shift1/15(dout14) -> fft_core1/16
  a0p0_1st_shift1/16(dout15) -> fft_core1/17
  a0p0_1st_shift1/17(dout16) -> fft_core1/18
  Subsystem6/6(Out5) -> a0p0_1st_shift1/6(din5)
  Subsystem6/9(Out8) -> a0p0_1st_shift1/9(din8)
  Subsystem6/14(Out13) -> a0p0_1st_shift1/14(din13)
  Subsystem6/16(Out15) -> a0p0_1st_shift1/16(din15)
  Subsystem6/12(Out11) -> a0p0_1st_shift1/12(din11)
  Subsystem6/2(Out1) -> a0p0_1st_shift1/2(din1)
  Subsystem6/17(Out16) -> a0p0_1st_shift1/17(din16)
  Subsystem6/4(Out3) -> a0p0_1st_shift1/4(din3)
  Subsystem6/10(Out9) -> a0p0_1st_shift1/10(din9)
  Subsystem6/7(Out6) -> a0p0_1st_shift1/7(din6)
  Subsystem6/5(Out4) -> a0p0_1st_shift1/5(din4)
  Subsystem6/13(Out12) -> a0p0_1st_shift1/13(din12)
  Subsystem6/8(Out7) -> a0p0_1st_shift1/8(din7)
  Subsystem6/1(sync_out) -> a0p0_1st_shift1/1(sync_in)
  Subsystem6/3(Out2) -> a0p0_1st_shift1/3(din2)
  Subsystem6/15(Out14) -> a0p0_1st_shift1/15(din14)
  Subsystem6/11(Out10) -> a0p0_1st_shift1/11(din10)
  fir_1/10 -> Subsystem6/10(In9)
  fir_1/11 -> Subsystem6/11(In10)
  fir_1/12 -> Subsystem6/12(In11)
  fir_1/2 -> pipeline93/1(d), Subsystem6/2(In1)
  fir_1/3 -> Subsystem6/3(In2)
  fir_1/4 -> Subsystem6/4(In3)
  fir_1/5 -> Subsystem6/5(In4)
  fir_1/13 -> Subsystem6/13(In12)
  fir_1/14 -> Subsystem6/14(In13)
  fir_1/15 -> Subsystem6/15(In14)
  fir_1/6 -> Subsystem6/6(In5)
  fir_1/7 -> Subsystem6/7(In6)
  fir_1/8 -> Subsystem6/8(In7)
  fir_1/16 -> Subsystem6/16(In15)
  fir_1/17 -> Subsystem6/17(In16)
  fir_1/9 -> Subsystem6/9(In8)
  fir_1/1 -> Subsystem6/1(sync)
  fft_core0/1 -> pipeline49/1(d)
  fft_core0/2 -> pipeline50/1(d)
  fft_core0/3 -> pipeline51/1(d)
  fft_core0/4 -> pipeline52/1(d)
  fft_core0/5 -> pipeline53/1(d)
  fft_core0/6 -> pipeline54/1(d)
  fft_core0/7 -> pipeline55/1(d)
  fft_core0/8 -> pipeline56/1(d)
  fft_core0/9 -> pipeline57/1(d)
  fft_core0/10 -> pipeline58/1(d)
  fft_core1/5 -> pipeline63/1(d)
  fft_core1/4 -> pipeline62/1(d)
  fft_core1/3 -> pipeline61/1(d)
  fft_core1/2 -> c_to_ri1/1, pipeline60/1(d)
  fft_core1/6 -> pipeline64/1(d)
  fft_core1/7 -> pipeline65/1(d)
  fft_core1/8 -> pipeline66/1(d)
  fft_core1/9 -> pipeline67/1(d)
  fft_core1/10 -> pipeline68/1(d)
  addtree1/1(sync_out) -> sync_gen1/1(sync), edge_detect7/1(in)
  addtree1/2(dout00) -> Reinterpret/1
  addtree1/3(dout11) -> Reinterpret1/1
  Reinterpret3/1 -> Convert9/1
  Convert9/1 -> pipeline85/1(d)
  simple_bram_vacc3/2(valid) -> edge_detect6/1(in), pipeline69/1(d)
  edge_detect6/1(out) -> corr01_i/3(trig)
  simple_bram_vacc3/1(dout) -> pipeline70/1(d)
  pipeline69/1(q) -> corr01_i/2(we)
  pipeline70/1(q) -> corr01_i/1(din)
  pipeline71/1(q) -> simple_bram_vacc3/1(new_acc)
  pipeline72/1(q) -> simple_bram_vacc3/2(din)
  addtree1/4(dout01) -> c_to_ri/1
  c_to_ri/1 -> Reinterpret2/1
  c_to_ri/2 -> Reinterpret3/1
  pipeline73/1(q) -> Slice14/1
  pipeline74/1(q) -> Slice6/1
  pipeline38/1(q) -> Counter3/2
  pipeline76/1(q) -> Counter1/1
  pipeline77/1(q) -> Register19/2
  pipeline75/1(q) -> Slice1/1, Slice/1
  [mrst] -> packetiser/2(mrst_in)
  edge_detect7/1(out) -> packetiser/1(sync_in)
  packetiser/1(mcnt_out) -> pipeline87/1(d)
  Register1/1 -> Slice26/1, Slice29/1
  Slice26/1 -> pipeline80/1(d)
  Slice29/1 -> pipeline86/1(d)
  transpose2/1(sync_out) -> [reorder0_sync]
  transpose2/2(dout) -> [reorder_data0]
  transpose1/2(dout) -> [reorder_data1]
  transpose1/1(sync_out) -> [reorder1_sync]
  acc_len/1(in_reg) -> sync_gen1/2(acc_len)
  pipeline82/1(q) -> pipeline26/1(d)
  pipeline84/1(q) -> pipeline30/1(d)
  pipeline85/1(q) -> pipeline72/1(d)
  pipeline87/1(q) -> Register1/1
  roach_gpioa6/1 -> pipeline88/1(d)
  roach_gpioa7/1 -> pipeline91/1(d)
  arm13/1 -> Delay1/1(d)
  [ps_en] -> Logical/1
  Logical/1 -> do_not_fan_out/1(d)
  Logical5/1 -> do_not_fan_out1/1(d)
  [ps_en] -> Logical5/2
  [adc0_ps] -> phase_invert2/1(invert)
  pipeline13/1(q) -> phase_invert2/2(din)
  phase_invert2/1(dout) -> [adc0]
  pipeline11/1(q) -> phase_invert1/2(din)
  phase_invert1/1(dout) -> [adc1]
  [adc1_ps] -> phase_invert1/1(invert)
  Delay1/1(q) -> [ps_en]
  pipeline88/1(q) -> Logical/2, [adc0_ps_gpio]
  do_not_fan_out/1(q) -> [adc0_ps]
  do_not_fan_out1/1(q) -> [adc1_ps]
  pipeline91/1(q) -> Logical5/1, [adc1_ps_gpio]
  bus_expand4/2(lsb_out1) -> delay_gen1/7(din0)
  bus_expand4/1(msb_out2) -> delay_gen1/1(sync_in)
  cd_tr1/5(dout) -> bus_expand4/1(bus_in)
  [sync] -> Concat3/1
  [data_adc1] -> Concat3/2
  Concat3/1 -> cd_tr1/7(din)
  adc5g_0/1(a0) -> conv_obbus_0/1(i0)
  adc5g_0/2(a1) -> conv_obbus_0/2(i1)
  adc5g_0/3(a2) -> conv_obbus_0/3(i2)
  adc5g_0/4(a3) -> conv_obbus_0/4(i3)
  adc5g_0/5(a4) -> conv_obbus_0/5(i4)
  adc5g_0/6(a5) -> conv_obbus_0/6(i5)
  adc5g_0/7(a6) -> conv_obbus_0/7(i6)
  adc5g_0/8(a7) -> conv_obbus_0/8(i7)
  adc5g_0/9(a8) -> conv_obbus_0/9(i8)
  adc5g_0/10(a9) -> conv_obbus_0/10(i9)
  adc5g_0/11(a10) -> conv_obbus_0/11(i10)
  adc5g_0/12(a11) -> conv_obbus_0/12(i11)
  adc5g_0/13(a12) -> conv_obbus_0/13(i12)
  adc5g_0/14(a13) -> conv_obbus_0/14(i13)
  adc5g_0/15(a14) -> conv_obbus_0/15(i14)
  adc5g_0/16(a15) -> conv_obbus_0/16(i15)
  conv_obbus_0/14(q13) -> bus_create2/14(in14)
  conv_obbus_0/12(q11) -> bus_create2/12(in12)
  conv_obbus_0/10(q9) -> bus_create2/10(in10)
  conv_obbus_0/11(q10) -> bus_create2/11(in11)
  conv_obbus_0/15(q14) -> bus_create2/15(in15)
  conv_obbus_0/13(q12) -> bus_create2/13(in13)
  conv_obbus_0/16(q15) -> bus_create2/16(in16)
  conv_obbus_0/1(q0) -> bus_create2/1(in1)
  conv_obbus_0/2(q1) -> bus_create2/2(in2)
  conv_obbus_0/3(q2) -> bus_create2/3(in3)
  conv_obbus_0/4(q3) -> bus_create2/4(in4)
  conv_obbus_0/5(q4) -> bus_create2/5(in5)
  conv_obbus_0/6(q5) -> bus_create2/6(in6)
  conv_obbus_0/7(q6) -> bus_create2/7(in7)
  conv_obbus_0/8(q7) -> bus_create2/8(in8)
  conv_obbus_0/9(q8) -> bus_create2/9(in9)
  adc5g_1/1(a0) -> conv_obbus_1/1(i0)
  adc5g_1/2(a1) -> conv_obbus_1/2(i1)
  adc5g_1/3(a2) -> conv_obbus_1/3(i2)
  adc5g_1/4(a3) -> conv_obbus_1/4(i3)
  adc5g_1/5(a4) -> conv_obbus_1/5(i4)
  adc5g_1/6(a5) -> conv_obbus_1/6(i5)
  adc5g_1/7(a6) -> conv_obbus_1/7(i6)
  adc5g_1/8(a7) -> conv_obbus_1/8(i7)
  adc5g_1/9(a8) -> conv_obbus_1/9(i8)
  adc5g_1/10(a9) -> conv_obbus_1/10(i9)
  adc5g_1/11(a10) -> conv_obbus_1/11(i10)
  adc5g_1/12(a11) -> conv_obbus_1/12(i11)
  adc5g_1/13(a12) -> conv_obbus_1/13(i12)
  adc5g_1/14(a13) -> conv_obbus_1/14(i13)
  adc5g_1/15(a14) -> conv_obbus_1/15(i14)
  adc5g_1/16(a15) -> conv_obbus_1/16(i15)
  conv_obbus_1/15(q14) -> bus_create3/15(in15)
  conv_obbus_1/16(q15) -> bus_create3/16(in16)
  conv_obbus_1/1(q0) -> bus_create3/1(in1)
  conv_obbus_1/2(q1) -> bus_create3/2(in2)
  conv_obbus_1/3(q2) -> bus_create3/3(in3)
  conv_obbus_1/4(q3) -> bus_create3/4(in4)
  conv_obbus_1/5(q4) -> bus_create3/5(in5)
  conv_obbus_1/6(q5) -> bus_create3/6(in6)
  conv_obbus_1/7(q6) -> bus_create3/7(in7)
  conv_obbus_1/8(q7) -> bus_create3/8(in8)
  conv_obbus_1/9(q8) -> bus_create3/9(in9)
  conv_obbus_1/10(q9) -> bus_create3/10(in10)
  conv_obbus_1/11(q10) -> bus_create3/11(in11)
  conv_obbus_1/12(q11) -> bus_create3/12(in12)
  conv_obbus_1/13(q12) -> bus_create3/13(in13)
  conv_obbus_1/14(q13) -> bus_create3/14(in14)
  [adc_sync0] -> pipeline89/1(d)
  pipeline89/1(q) -> snapshot_adc0/3(trig)
  Constant55/1 -> snapshot_adc0/2(we)
  [adc1] -> pipeline44/1(d)
  pipeline44/1(q) -> snapshot_adc1/1(din)
  [adc_sync0] -> pipeline90/1(d)
  pipeline90/1(q) -> snapshot_adc1/3(trig)
  Constant56/1 -> snapshot_adc1/2(we)
  pipeline46/1(q) -> [quant1_sync]
  fine_del0/2 -> pipeline78/1(d)
  pipeline79/1(q) -> [quant0_sync]
  pipeline33/1(q) -> cross_multiplier/3(din1)
  pipeline32/1(q) -> cross_multiplier/2(din0)
  pipeline31/1(q) -> cross_multiplier/1(sync_in)
  cross_multiplier/1(sync_out) -> pipeline34/1(d)
  cross_multiplier/2(din0_x_din0*) -> pipeline35/1(d)
  cross_multiplier/4(din1_x_din1*) -> pipeline36/1(d)
  cross_multiplier/3(din0_x_din1*) -> pipeline37/1(d)
  pipeline80/1(q) -> mcnt_lsb/1(out_reg)
  pipeline86/1(q) -> cast_gw/1
  cast_gw/1 -> mcnt_msb/1(out_reg)
  delay_0/1 -> reint/1(sync)
  delay_0/2 -> reint/2(i0)
  delay_0/3 -> reint/3(i1)
  delay_0/4 -> reint/4(i2)
  delay_0/5 -> reint/5(i3)
  delay_0/6 -> reint/6(i4)
  delay_0/7 -> reint/7(i5)
  delay_0/8 -> reint/8(i6)
  delay_0/9 -> reint/9(i7)
  delay_0/10 -> reint/10(i8)
  delay_0/11 -> reint/11(i9)
  delay_0/12 -> reint/12(i10)
  delay_0/13 -> reint/13(i11)
  delay_0/14 -> reint/14(i12)
  delay_0/15 -> reint/15(i13)
  delay_0/16 -> reint/16(i14)
  delay_0/17 -> reint/17(i15)
  reint/1(sync_out) -> Subsystem2/1(sync)
  reint/10(q8) -> Subsystem2/10(In9)
  reint/11(q9) -> Subsystem2/11(In10)
  reint/7(q5) -> Subsystem2/7(In6)
  reint/12(q10) -> Subsystem2/12(In11)
  reint/13(q11) -> Subsystem2/13(In12)
  reint/14(q12) -> Subsystem2/14(In13)
  reint/15(q13) -> Subsystem2/15(In14)
  reint/16(q14) -> Subsystem2/16(In15)
  reint/17(q15) -> Subsystem2/17(In16)
  reint/4(q2) -> Subsystem2/4(In3)
  reint/6(q4) -> Subsystem2/6(In5)
  reint/3(q1) -> Subsystem2/3(In2)
  reint/8(q6) -> Subsystem2/8(In7)
  reint/2(q0) -> Subsystem2/2(In1)
  reint/5(q3) -> Subsystem2/5(In4)
  reint/9(q7) -> Subsystem2/9(In8)
  delay_1/1 -> reint1/1(sync)
  delay_1/2 -> pipeline92/1(d), reint1/2(i0)
  delay_1/3 -> reint1/3(i1)
  delay_1/4 -> reint1/4(i2)
  delay_1/5 -> reint1/5(i3)
  delay_1/6 -> reint1/6(i4)
  delay_1/7 -> reint1/7(i5)
  delay_1/8 -> reint1/8(i6)
  delay_1/9 -> reint1/9(i7)
  delay_1/10 -> reint1/10(i8)
  delay_1/11 -> reint1/11(i9)
  delay_1/12 -> reint1/12(i10)
  delay_1/13 -> reint1/13(i11)
  delay_1/14 -> reint1/14(i12)
  delay_1/15 -> reint1/15(i13)
  delay_1/16 -> reint1/16(i14)
  delay_1/17 -> reint1/17(i15)
  reint1/1(sync_out) -> Subsystem3/1(sync)
  reint1/10(q8) -> Subsystem3/10(In9)
  reint1/11(q9) -> Subsystem3/11(In10)
  reint1/12(q10) -> Subsystem3/12(In11)
  reint1/2(q0) -> Subsystem3/2(In1)
  reint1/3(q1) -> Subsystem3/3(In2)
  reint1/4(q2) -> Subsystem3/4(In3)
  reint1/5(q3) -> Subsystem3/5(In4)
  reint1/6(q4) -> Subsystem3/6(In5)
  reint1/7(q5) -> Subsystem3/7(In6)
  reint1/8(q6) -> Subsystem3/8(In7)
  reint1/13(q11) -> Subsystem3/13(In12)
  reint1/14(q12) -> Subsystem3/14(In13)
  reint1/15(q13) -> Subsystem3/15(In14)
  reint1/16(q14) -> Subsystem3/16(In15)
  reint1/17(q15) -> Subsystem3/17(In16)
  reint1/9(q7) -> Subsystem3/9(In8)
  Constant30/1 -> snapshot_fft_r1/2(we)
  Constant46/1 -> snapshot_fir1/2(we)
  Constant41/1 -> snapshot_fir1/3(trig)
  Constant57/1 -> snapshot_delay1/3(trig)
  Constant58/1 -> snapshot_delay1/2(we)
  pipeline92/1(q) -> snapshot_delay1/1(din)
  pipeline93/1(q) -> snapshot_fir1/1(din)
  pipeline94/1(q) -> snapshot_fft_r1/1(din)
  Constant59/1 -> snapshot_fft_in1/3(trig)
  Constant60/1 -> snapshot_fft_in1/2(we)
  pipeline95/1(q) -> snapshot_fft_in1/1(din)
  fft_core1/1 -> pipeline102/1(d), pipeline101/1(d), pipeline59/1(d)
  Constant62/1 -> snapshot_fft_i1/2(we)
  pipeline96/1(q) -> snapshot_fft_i1/1(din)
  c_to_ri1/1 -> pipeline94/1(d)
  c_to_ri1/2 -> pipeline96/1(d)
  Constant64/1 -> snapshot_fd_r1/2(we)
  pipeline97/1(q) -> snapshot_fd_r1/1(din)
  fine_del1/1 -> pipeline104/1(d), pipeline103/1(d), pipeline46/1(d)
  Constant66/1 -> snapshot_fd_im1/2(we)
  pipeline98/1(q) -> snapshot_fd_im1/1(din)
  c_to_ri2/1 -> pipeline97/1(d)
  c_to_ri2/2 -> pipeline98/1(d)
  Slice30/1 -> c_to_ri2/1
  Constant63/1 -> snapshot_pre_vacc/2(we)
  pipeline99/1(q) -> snapshot_pre_vacc/1(din)
  sync_gen1/1(sync_out) -> Register1/2, pipeline25/1(d), pipeline27/1(d), pipeline100/1(d), pipeline71/1(d), pipeline29/1(d)
  pipeline83/1(q) -> pipeline99/1(d), pipeline28/1(d)
  pipeline100/1(q) -> snapshot_pre_vacc/3(trig)
  pipeline101/1(q) -> snapshot_fft_r1/3(trig)
  pipeline102/1(q) -> snapshot_fft_i1/3(trig)
  pipeline103/1(q) -> snapshot_fd_r1/3(trig)
  pipeline104/1(q) -> snapshot_fd_im1/3(trig)
  pipeline105/1(q) -> delay_tr_status1/1(reg_out)
  pipeline106/1(q) -> delay_tr_status0/1(reg_out)
  pipeline107/1(q) -> fd_tr0/2(load_now)
  pipeline108/1(q) -> fd_tr0/3(arm)
  pipeline109/1(q) -> fd_tr1/2(load_now)
  pipeline110/1(q) -> fd_tr1/3(arm)
